simulink model "Test_Display"  (Simulink 8.1)
settings: Solver=ode45  SolverMode=SingleTasking  StartTime=0.0  StopTime=10.0  RelTol=1e-3
undefined symbols (not defined in the file): get, hot
libraries: dspsnks4 x1
(part 2 of 3)

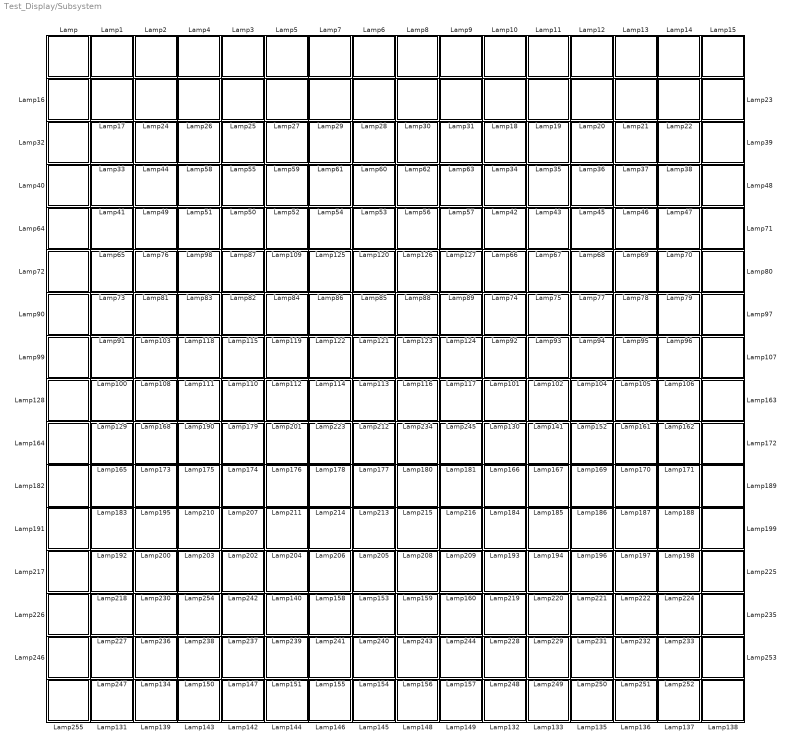
== system Test_Display/Subsystem ==
  Lamp : Subsystem  DialogController=hmiCreateDDGDialog  mask(MWDashboardBlock){webBlockId=edf84850-d0fe-4c8a-86f7-eea0c37b674f, webBlockType=lamp, ShowInLibBrowser=on, ShowInitialText=on, HMISrcModelName=[]}
      mask prompts: webBlockType "WebBlock Type"; HMISrcModelName "Source Model"
      mask Help: helpview([docroot '/mapfiles/simulink.map'], 'hmi_lamp')
      mask Display:
      | if strcmp(get_param(bdroot(gcb),'BlockDiagramType'), 'library')
      |     image([(matlabroot) '/toolbox/simulink/hmi/icons/Lamp.png']);
      | end
  Lamp1 : Subsystem  DialogController=hmiCreateDDGDialog  mask(MWDashboardBlock){webBlockId=fd4cb8b6-599e-465c-bf44-31615dcb3fd4, webBlockType=lamp, ShowInLibBrowser=on, ShowInitialText=on, HMISrcModelName=[]}
      mask prompts: webBlockType "WebBlock Type"; HMISrcModelName "Source Model"
      mask Help: helpview([docroot '/mapfiles/simulink.map'], 'hmi_lamp')
      mask Display:
      | if strcmp(get_param(bdroot(gcb),'BlockDiagramType'), 'library')
      |     image([(matlabroot) '/toolbox/simulink/hmi/icons/Lamp.png']);
      | end
  Lamp10 : Subsystem  DialogController=hmiCreateDDGDialog  mask(MWDashboardBlock){webBlockId=69970134-2694-491f-b422-9ae462ee0038, webBlockType=lamp, ShowInLibBrowser=on, ShowInitialText=on, HMISrcModelName=[]}
      mask prompts: webBlockType "WebBlock Type"; HMISrcModelName "Source Model"
      mask Help: helpview([docroot '/mapfiles/simulink.map'], 'hmi_lamp')
      mask Display:
      | if strcmp(get_param(bdroot(gcb),'BlockDiagramType'), 'library')
      |     image([(matlabroot) '/toolbox/simulink/hmi/icons/Lamp.png']);
      | end
  Lamp100 : Subsystem  DialogController=hmiCreateDDGDialog  mask(MWDashboardBlock){webBlockId=49397023-e76e-4e1f-be5b-ec227a720212, webBlockType=lamp, ShowInLibBrowser=on, ShowInitialText=on, HMISrcModelName=[]}
      mask prompts: webBlockType "WebBlock Type"; HMISrcModelName "Source Model"
      mask Help: helpview([docroot '/mapfiles/simulink.map'], 'hmi_lamp')
      mask Display:
      | if strcmp(get_param(bdroot(gcb),'BlockDiagramType'), 'library')
      |     image([(matlabroot) '/toolbox/simulink/hmi/icons/Lamp.png']);
      | end
  Lamp101 : Subsystem  DialogController=hmiCreateDDGDialog  mask(MWDashboardBlock){webBlockId=21b2a518-b5e8-4574-abab-928d7426710c, webBlockType=lamp, ShowInLibBrowser=on, ShowInitialText=on, HMISrcModelName=[]}
      mask prompts: webBlockType "WebBlock Type"; HMISrcModelName "Source Model"
      mask Help: helpview([docroot '/mapfiles/simulink.map'], 'hmi_lamp')
      mask Display:
      | if strcmp(get_param(bdroot(gcb),'BlockDiagramType'), 'library')
      |     image([(matlabroot) '/toolbox/simulink/hmi/icons/Lamp.png']);
      | end
  Lamp102 : Subsystem  DialogController=hmiCreateDDGDialog  mask(MWDashboardBlock){webBlockId=9ad93c2d-efff-4ac7-a816-7961f3646538, webBlockType=lamp, ShowInLibBrowser=on, ShowInitialText=on, HMISrcModelName=[]}
      mask prompts: webBlockType "WebBlock Type"; HMISrcModelName "Source Model"
      mask Help: helpview([docroot '/mapfiles/simulink.map'], 'hmi_lamp')
      mask Display:
      | if strcmp(get_param(bdroot(gcb),'BlockDiagramType'), 'library')
      |     image([(matlabroot) '/toolbox/simulink/hmi/icons/Lamp.png']);
      | end
  Lamp103 : Subsystem  DialogController=hmiCreateDDGDialog  mask(MWDashboardBlock){webBlockId=b3c12dab-38df-4fcb-add2-5a3df45dc055, webBlockType=lamp, ShowInLibBrowser=on, ShowInitialText=on, HMISrcModelName=[]}
      mask prompts: webBlockType "WebBlock Type"; HMISrcModelName "Source Model"
      mask Help: helpview([docroot '/mapfiles/simulink.map'], 'hmi_lamp')
      mask Display:
      | if strcmp(get_param(bdroot(gcb),'BlockDiagramType'), 'library')
      |     image([(matlabroot) '/toolbox/simulink/hmi/icons/Lamp.png']);
      | end
  Lamp104 : Subsystem  DialogController=hmiCreateDDGDialog  mask(MWDashboardBlock){webBlockId=22654bdc-6924-4c41-873f-0dac80d459c9, webBlockType=lamp, ShowInLibBrowser=on, ShowInitialText=on, HMISrcModelName=[]}
      mask prompts: webBlockType "WebBlock Type"; HMISrcModelName "Source Model"
      mask Help: helpview([docroot '/mapfiles/simulink.map'], 'hmi_lamp')
      mask Display:
      | if strcmp(get_param(bdroot(gcb),'BlockDiagramType'), 'library')
      |     image([(matlabroot) '/toolbox/simulink/hmi/icons/Lamp.png']);
      | end
  Lamp105 : Subsystem  DialogController=hmiCreateDDGDialog  mask(MWDashboardBlock){webBlockId=5a7a78fc-d4e3-496d-b8a8-b493089be8de, webBlockType=lamp, ShowInLibBrowser=on, ShowInitialText=on, HMISrcModelName=[]}
      mask prompts: webBlockType "WebBlock Type"; HMISrcModelName "Source Model"
      mask Help: helpview([docroot '/mapfiles/simulink.map'], 'hmi_lamp')
      mask Display:
      | if strcmp(get_param(bdroot(gcb),'BlockDiagramType'), 'library')
      |     image([(matlabroot) '/toolbox/simulink/hmi/icons/Lamp.png']);
      | end
  Lamp106 : Subsystem  DialogController=hmiCreateDDGDialog  mask(MWDashboardBlock){webBlockId=3a2bc532-a839-46f6-9bbc-20018f0d8f64, webBlockType=lamp, ShowInLibBrowser=on, ShowInitialText=on, HMISrcModelName=[]}
      mask prompts: webBlockType "WebBlock Type"; HMISrcModelName "Source Model"
      mask Help: helpview([docroot '/mapfiles/simulink.map'], 'hmi_lamp')
      mask Display:
      | if strcmp(get_param(bdroot(gcb),'BlockDiagramType'), 'library')
      |     image([(matlabroot) '/toolbox/simulink/hmi/icons/Lamp.png']);
      | end
  Lamp107 : Subsystem  DialogController=hmiCreateDDGDialog  mask(MWDashboardBlock){webBlockId=dba8c154-a909-43bc-b6e3-c0b3528fa1e0, webBlockType=lamp, ShowInLibBrowser=on, ShowInitialText=on, HMISrcModelName=[]}
      mask prompts: webBlockType "WebBlock Type"; HMISrcModelName "Source Model"
      mask Help: helpview([docroot '/mapfiles/simulink.map'], 'hmi_lamp')
      mask Display:
      | if strcmp(get_param(bdroot(gcb),'BlockDiagramType'), 'library')
      |     image([(matlabroot) '/toolbox/simulink/hmi/icons/Lamp.png']);
      | end
  Lamp108 : Subsystem  DialogController=hmiCreateDDGDialog  mask(MWDashboardBlock){webBlockId=a7c0c051-3ddd-4c85-a3d7-890d827bbacd, webBlockType=lamp, ShowInLibBrowser=on, ShowInitialText=on, HMISrcModelName=[]}
      mask prompts: webBlockType "WebBlock Type"; HMISrcModelName "Source Model"
      mask Help: helpview([docroot '/mapfiles/simulink.map'], 'hmi_lamp')
      mask Display:
      | if strcmp(get_param(bdroot(gcb),'BlockDiagramType'), 'library')
      |     image([(matlabroot) '/toolbox/simulink/hmi/icons/Lamp.png']);
      | end
  Lamp109 : Subsystem  DialogController=hmiCreateDDGDialog  mask(MWDashboardBlock){webBlockId=68039627-b65d-475a-b7d3-5dd921e9c6da, webBlockType=lamp, ShowInLibBrowser=on, ShowInitialText=on, HMISrcModelName=[]}
      mask prompts: webBlockType "WebBlock Type"; HMISrcModelName "Source Model"
      mask Help: helpview([docroot '/mapfiles/simulink.map'], 'hmi_lamp')
      mask Display:
      | if strcmp(get_param(bdroot(gcb),'BlockDiagramType'), 'library')
      |     image([(matlabroot) '/toolbox/simulink/hmi/icons/Lamp.png']);
      | end
  Lamp11 : Subsystem  DialogController=hmiCreateDDGDialog  mask(MWDashboardBlock){webBlockId=17d759d2-7a4a-42db-8b8d-8621e0edc736, webBlockType=lamp, ShowInLibBrowser=on, ShowInitialText=on, HMISrcModelName=[]}
      mask prompts: webBlockType "WebBlock Type"; HMISrcModelName "Source Model"
      mask Help: helpview([docroot '/mapfiles/simulink.map'], 'hmi_lamp')
      mask Display:
      | if strcmp(get_param(bdroot(gcb),'BlockDiagramType'), 'library')
      |     image([(matlabroot) '/toolbox/simulink/hmi/icons/Lamp.png']);
      | end
  Lamp110 : Subsystem  DialogController=hmiCreateDDGDialog  mask(MWDashboardBlock){webBlockId=ad71e308-a508-459b-8e0f-4282464f22fe, webBlockType=lamp, ShowInLibBrowser=on, ShowInitialText=on, HMISrcModelName=[]}
      mask prompts: webBlockType "WebBlock Type"; HMISrcModelName "Source Model"
      mask Help: helpview([docroot '/mapfiles/simulink.map'], 'hmi_lamp')
      mask Display:
      | if strcmp(get_param(bdroot(gcb),'BlockDiagramType'), 'library')
      |     image([(matlabroot) '/toolbox/simulink/hmi/icons/Lamp.png']);
      | end
  Lamp111 : Subsystem  DialogController=hmiCreateDDGDialog  mask(MWDashboardBlock){webBlockId=650bb823-101c-407e-9790-47f3807fb796, webBlockType=lamp, ShowInLibBrowser=on, ShowInitialText=on, HMISrcModelName=[]}
      mask prompts: webBlockType "WebBlock Type"; HMISrcModelName "Source Model"
      mask Help: helpview([docroot '/mapfiles/simulink.map'], 'hmi_lamp')
      mask Display:
      | if strcmp(get_param(bdroot(gcb),'BlockDiagramType'), 'library')
      |     image([(matlabroot) '/toolbox/simulink/hmi/icons/Lamp.png']);
      | end
  Lamp112 : Subsystem  DialogController=hmiCreateDDGDialog  mask(MWDashboardBlock){webBlockId=423ee99d-c28c-43df-a12a-3af234ac6943, webBlockType=lamp, ShowInLibBrowser=on, ShowInitialText=on, HMISrcModelName=[]}
      mask prompts: webBlockType "WebBlock Type"; HMISrcModelName "Source Model"
      mask Help: helpview([docroot '/mapfiles/simulink.map'], 'hmi_lamp')
      mask Display:
      | if strcmp(get_param(bdroot(gcb),'BlockDiagramType'), 'library')
      |     image([(matlabroot) '/toolbox/simulink/hmi/icons/Lamp.png']);
      | end
  Lamp113 : Subsystem  DialogController=hmiCreateDDGDialog  mask(MWDashboardBlock){webBlockId=1a9c237c-8958-40c1-8183-6b5bf75441e2, webBlockType=lamp, ShowInLibBrowser=on, ShowInitialText=on, HMISrcModelName=[]}
      mask prompts: webBlockType "WebBlock Type"; HMISrcModelName "Source Model"
      mask Help: helpview([docroot '/mapfiles/simulink.map'], 'hmi_lamp')
      mask Display:
      | if strcmp(get_param(bdroot(gcb),'BlockDiagramType'), 'library')
      |     image([(matlabroot) '/toolbox/simulink/hmi/icons/Lamp.png']);
      | end
  Lamp114 : Subsystem  DialogController=hmiCreateDDGDialog  mask(MWDashboardBlock){webBlockId=59713dff-163f-48a3-89de-46bb5d4dd39c, webBlockType=lamp, ShowInLibBrowser=on, ShowInitialText=on, HMISrcModelName=[]}
      mask prompts: webBlockType "WebBlock Type"; HMISrcModelName "Source Model"
      mask Help: helpview([docroot '/mapfiles/simulink.map'], 'hmi_lamp')
      mask Display:
      | if strcmp(get_param(bdroot(gcb),'BlockDiagramType'), 'library')
      |     image([(matlabroot) '/toolbox/simulink/hmi/icons/Lamp.png']);
      | end
  Lamp115 : Subsystem  DialogController=hmiCreateDDGDialog  mask(MWDashboardBlock){webBlockId=ca91e4aa-4a84-4aef-8eff-59d3ab8b4ed0, webBlockType=lamp, ShowInLibBrowser=on, ShowInitialText=on, HMISrcModelName=[]}
      mask prompts: webBlockType "WebBlock Type"; HMISrcModelName "Source Model"
      mask Help: helpview([docroot '/mapfiles/simulink.map'], 'hmi_lamp')
      mask Display:
      | if strcmp(get_param(bdroot(gcb),'BlockDiagramType'), 'library')
      |     image([(matlabroot) '/toolbox/simulink/hmi/icons/Lamp.png']);
      | end
  Lamp116 : Subsystem  DialogController=hmiCreateDDGDialog  mask(MWDashboardBlock){webBlockId=ea0446a5-980a-44d1-baf7-efdbd4c4c0cf, webBlockType=lamp, ShowInLibBrowser=on, ShowInitialText=on, HMISrcModelName=[]}
      mask prompts: webBlockType "WebBlock Type"; HMISrcModelName "Source Model"
      mask Help: helpview([docroot '/mapfiles/simulink.map'], 'hmi_lamp')
      mask Display:
      | if strcmp(get_param(bdroot(gcb),'BlockDiagramType'), 'library')
      |     image([(matlabroot) '/toolbox/simulink/hmi/icons/Lamp.png']);
      | end
  Lamp117 : Subsystem  DialogController=hmiCreateDDGDialog  mask(MWDashboardBlock){webBlockId=6f6da4d9-b8fd-41db-ad2e-5eafed5489c3, webBlockType=lamp, ShowInLibBrowser=on, ShowInitialText=on, HMISrcModelName=[]}
      mask prompts: webBlockType "WebBlock Type"; HMISrcModelName "Source Model"
      mask Help: helpview([docroot '/mapfiles/simulink.map'], 'hmi_lamp')
      mask Display:
      | if strcmp(get_param(bdroot(gcb),'BlockDiagramType'), 'library')
      |     image([(matlabroot) '/toolbox/simulink/hmi/icons/Lamp.png']);
      | end
  Lamp118 : Subsystem  DialogController=hmiCreateDDGDialog  mask(MWDashboardBlock){webBlockId=a4cd4763-fce0-4138-a61c-a9eaa5240dcf, webBlockType=lamp, ShowInLibBrowser=on, ShowInitialText=on, HMISrcModelName=[]}
      mask prompts: webBlockType "WebBlock Type"; HMISrcModelName "Source Model"
      mask Help: helpview([docroot '/mapfiles/simulink.map'], 'hmi_lamp')
      mask Display:
      | if strcmp(get_param(bdroot(gcb),'BlockDiagramType'), 'library')
      |     image([(matlabroot) '/toolbox/simulink/hmi/icons/Lamp.png']);
      | end
  Lamp119 : Subsystem  DialogController=hmiCreateDDGDialog  mask(MWDashboardBlock){webBlockId=e5efb401-ac08-44a6-bfd0-4540585fee9a, webBlockType=lamp, ShowInLibBrowser=on, ShowInitialText=on, HMISrcModelName=[]}
      mask prompts: webBlockType "WebBlock Type"; HMISrcModelName "Source Model"
      mask Help: helpview([docroot '/mapfiles/simulink.map'], 'hmi_lamp')
      mask Display:
      | if strcmp(get_param(bdroot(gcb),'BlockDiagramType'), 'library')
      |     image([(matlabroot) '/toolbox/simulink/hmi/icons/Lamp.png']);
      | end
  Lamp12 : Subsystem  DialogController=hmiCreateDDGDialog  mask(MWDashboardBlock){webBlockId=2739aeb3-55c9-4fba-ad1b-ffe4ed783479, webBlockType=lamp, ShowInLibBrowser=on, ShowInitialText=on, HMISrcModelName=[]}
      mask prompts: webBlockType "WebBlock Type"; HMISrcModelName "Source Model"
      mask Help: helpview([docroot '/mapfiles/simulink.map'], 'hmi_lamp')
      mask Display:
      | if strcmp(get_param(bdroot(gcb),'BlockDiagramType'), 'library')
      |     image([(matlabroot) '/toolbox/simulink/hmi/icons/Lamp.png']);
      | end
  Lamp120 : Subsystem  DialogController=hmiCreateDDGDialog  mask(MWDashboardBlock){webBlockId=4de6be70-ca78-43c6-a822-f9fd70f81b9a, webBlockType=lamp, ShowInLibBrowser=on, ShowInitialText=on, HMISrcModelName=[]}
      mask prompts: webBlockType "WebBlock Type"; HMISrcModelName "Source Model"
      mask Help: helpview([docroot '/mapfiles/simulink.map'], 'hmi_lamp')
      mask Display:
      | if strcmp(get_param(bdroot(gcb),'BlockDiagramType'), 'library')
      |     image([(matlabroot) '/toolbox/simulink/hmi/icons/Lamp.png']);
      | end
  Lamp121 : Subsystem  DialogController=hmiCreateDDGDialog  mask(MWDashboardBlock){webBlockId=ec3c07a6-ed4f-446b-a6db-729d5e1aac5e, webBlockType=lamp, ShowInLibBrowser=on, ShowInitialText=on, HMISrcModelName=[]}
      mask prompts: webBlockType "WebBlock Type"; HMISrcModelName "Source Model"
      mask Help: helpview([docroot '/mapfiles/simulink.map'], 'hmi_lamp')
      mask Display:
      | if strcmp(get_param(bdroot(gcb),'BlockDiagramType'), 'library')
      |     image([(matlabroot) '/toolbox/simulink/hmi/icons/Lamp.png']);
      | end
  Lamp122 : Subsystem  DialogController=hmiCreateDDGDialog  mask(MWDashboardBlock){webBlockId=6e468738-635a-42dc-b04e-3cbfa3067652, webBlockType=lamp, ShowInLibBrowser=on, ShowInitialText=on, HMISrcModelName=[]}
      mask prompts: webBlockType "WebBlock Type"; HMISrcModelName "Source Model"
      mask Help: helpview([docroot '/mapfiles/simulink.map'], 'hmi_lamp')
      mask Display:
      | if strcmp(get_param(bdroot(gcb),'BlockDiagramType'), 'library')
      |     image([(matlabroot) '/toolbox/simulink/hmi/icons/Lamp.png']);
      | end
  Lamp123 : Subsystem  DialogController=hmiCreateDDGDialog  mask(MWDashboardBlock){webBlockId=fb95ced1-5fd5-4dd6-99a4-486117cc7b04, webBlockType=lamp, ShowInLibBrowser=on, ShowInitialText=on, HMISrcModelName=[]}
      mask prompts: webBlockType "WebBlock Type"; HMISrcModelName "Source Model"
      mask Help: helpview([docroot '/mapfiles/simulink.map'], 'hmi_lamp')
      mask Display:
      | if strcmp(get_param(bdroot(gcb),'BlockDiagramType'), 'library')
      |     image([(matlabroot) '/toolbox/simulink/hmi/icons/Lamp.png']);
      | end
  Lamp124 : Subsystem  DialogController=hmiCreateDDGDialog  mask(MWDashboardBlock){webBlockId=8cc34a89-169c-45fb-add0-c245fffb35f4, webBlockType=lamp, ShowInLibBrowser=on, ShowInitialText=on, HMISrcModelName=[]}
      mask prompts: webBlockType "WebBlock Type"; HMISrcModelName "Source Model"
      mask Help: helpview([docroot '/mapfiles/simulink.map'], 'hmi_lamp')
      mask Display:
      | if strcmp(get_param(bdroot(gcb),'BlockDiagramType'), 'library')
      |     image([(matlabroot) '/toolbox/simulink/hmi/icons/Lamp.png']);
      | end
  Lamp125 : Subsystem  DialogController=hmiCreateDDGDialog  mask(MWDashboardBlock){webBlockId=5e75099f-bab6-47c8-9d5a-45cdd18ada81, webBlockType=lamp, ShowInLibBrowser=on, ShowInitialText=on, HMISrcModelName=[]}
      mask prompts: webBlockType "WebBlock Type"; HMISrcModelName "Source Model"
      mask Help: helpview([docroot '/mapfiles/simulink.map'], 'hmi_lamp')
      mask Display:
      | if strcmp(get_param(bdroot(gcb),'BlockDiagramType'), 'library')
      |     image([(matlabroot) '/toolbox/simulink/hmi/icons/Lamp.png']);
      | end
  Lamp126 : Subsystem  DialogController=hmiCreateDDGDialog  mask(MWDashboardBlock){webBlockId=b24af4a7-3b56-44e6-9307-9233d0605101, webBlockType=lamp, ShowInLibBrowser=on, ShowInitialText=on, HMISrcModelName=[]}
      mask prompts: webBlockType "WebBlock Type"; HMISrcModelName "Source Model"
      mask Help: helpview([docroot '/mapfiles/simulink.map'], 'hmi_lamp')
      mask Display:
      | if strcmp(get_param(bdroot(gcb),'BlockDiagramType'), 'library')
      |     image([(matlabroot) '/toolbox/simulink/hmi/icons/Lamp.png']);
      | end
  Lamp127 : Subsystem  DialogController=hmiCreateDDGDialog  mask(MWDashboardBlock){webBlockId=f9e12296-8670-4a96-b8dc-f227c20c59c8, webBlockType=lamp, ShowInLibBrowser=on, ShowInitialText=on, HMISrcModelName=[]}
      mask prompts: webBlockType "WebBlock Type"; HMISrcModelName "Source Model"
      mask Help: helpview([docroot '/mapfiles/simulink.map'], 'hmi_lamp')
      mask Display:
      | if strcmp(get_param(bdroot(gcb),'BlockDiagramType'), 'library')
      |     image([(matlabroot) '/toolbox/simulink/hmi/icons/Lamp.png']);
      | end
  Lamp128 : Subsystem  DialogController=hmiCreateDDGDialog  mask(MWDashboardBlock){webBlockId=639b4a5e-2d2b-4481-a81d-53f4802d670a, webBlockType=lamp, ShowInLibBrowser=on, ShowInitialText=on, HMISrcModelName=[]}
      mask prompts: webBlockType "WebBlock Type"; HMISrcModelName "Source Model"
      mask Help: helpview([docroot '/mapfiles/simulink.map'], 'hmi_lamp')
      mask Display:
      | if strcmp(get_param(bdroot(gcb),'BlockDiagramType'), 'library')
      |     image([(matlabroot) '/toolbox/simulink/hmi/icons/Lamp.png']);
      | end
  Lamp129 : Subsystem  DialogController=hmiCreateDDGDialog  mask(MWDashboardBlock){webBlockId=2bbac042-df92-44e2-886a-26cf5aa8e5a7, webBlockType=lamp, ShowInLibBrowser=on, ShowInitialText=on, HMISrcModelName=[]}
      mask prompts: webBlockType "WebBlock Type"; HMISrcModelName "Source Model"
      mask Help: helpview([docroot '/mapfiles/simulink.map'], 'hmi_lamp')
      mask Display:
      | if strcmp(get_param(bdroot(gcb),'BlockDiagramType'), 'library')
      |     image([(matlabroot) '/toolbox/simulink/hmi/icons/Lamp.png']);
      | end
  Lamp13 : Subsystem  DialogController=hmiCreateDDGDialog  mask(MWDashboardBlock){webBlockId=10de76a9-a845-4e5b-a06c-3d4b0e136d3c, webBlockType=lamp, ShowInLibBrowser=on, ShowInitialText=on, HMISrcModelName=[]}
      mask prompts: webBlockType "WebBlock Type"; HMISrcModelName "Source Model"
      mask Help: helpview([docroot '/mapfiles/simulink.map'], 'hmi_lamp')
      mask Display:
      | if strcmp(get_param(bdroot(gcb),'BlockDiagramType'), 'library')
      |     image([(matlabroot) '/toolbox/simulink/hmi/icons/Lamp.png']);
      | end
  Lamp130 : Subsystem  DialogController=hmiCreateDDGDialog  mask(MWDashboardBlock){webBlockId=03246cb9-1490-4c04-bce7-8577a1ad03d9, webBlockType=lamp, ShowInLibBrowser=on, ShowInitialText=on, HMISrcModelName=[]}
      mask prompts: webBlockType "WebBlock Type"; HMISrcModelName "Source Model"
      mask Help: helpview([docroot '/mapfiles/simulink.map'], 'hmi_lamp')
      mask Display:
      | if strcmp(get_param(bdroot(gcb),'BlockDiagramType'), 'library')
      |     image([(matlabroot) '/toolbox/simulink/hmi/icons/Lamp.png']);
      | end
  Lamp131 : Subsystem  DialogController=hmiCreateDDGDialog  mask(MWDashboardBlock){webBlockId=bc19434d-be49-4c90-9f4f-d30ae243e62e, webBlockType=lamp, ShowInLibBrowser=on, ShowInitialText=on, HMISrcModelName=[]}
      mask prompts: webBlockType "WebBlock Type"; HMISrcModelName "Source Model"
      mask Help: helpview([docroot '/mapfiles/simulink.map'], 'hmi_lamp')
      mask Display:
      | if strcmp(get_param(bdroot(gcb),'BlockDiagramType'), 'library')
      |     image([(matlabroot) '/toolbox/simulink/hmi/icons/Lamp.png']);
      | end
  Lamp132 : Subsystem  DialogController=hmiCreateDDGDialog  mask(MWDashboardBlock){webBlockId=69249e84-f16d-4676-be2b-d7059b0a9994, webBlockType=lamp, ShowInLibBrowser=on, ShowInitialText=on, HMISrcModelName=[]}
      mask prompts: webBlockType "WebBlock Type"; HMISrcModelName "Source Model"
      mask Help: helpview([docroot '/mapfiles/simulink.map'], 'hmi_lamp')
      mask Display:
      | if strcmp(get_param(bdroot(gcb),'BlockDiagramType'), 'library')
      |     image([(matlabroot) '/toolbox/simulink/hmi/icons/Lamp.png']);
      | end
  Lamp133 : Subsystem  DialogController=hmiCreateDDGDialog  mask(MWDashboardBlock){webBlockId=a551e0c3-b966-4766-ba83-f6a20ae4271b, webBlockType=lamp, ShowInLibBrowser=on, ShowInitialText=on, HMISrcModelName=[]}
      mask prompts: webBlockType "WebBlock Type"; HMISrcModelName "Source Model"
      mask Help: helpview([docroot '/mapfiles/simulink.map'], 'hmi_lamp')
      mask Display:
      | if strcmp(get_param(bdroot(gcb),'BlockDiagramType'), 'library')
      |     image([(matlabroot) '/toolbox/simulink/hmi/icons/Lamp.png']);
      | end
  Lamp134 : Subsystem  DialogController=hmiCreateDDGDialog  mask(MWDashboardBlock){webBlockId=9226dd28-2f61-4cbc-916d-2f003ff13875, webBlockType=lamp, ShowInLibBrowser=on, ShowInitialText=on, HMISrcModelName=[]}
      mask prompts: webBlockType "WebBlock Type"; HMISrcModelName "Source Model"
      mask Help: helpview([docroot '/mapfiles/simulink.map'], 'hmi_lamp')
      mask Display:
      | if strcmp(get_param(bdroot(gcb),'BlockDiagramType'), 'library')
      |     image([(matlabroot) '/toolbox/simulink/hmi/icons/Lamp.png']);
      | end
  Lamp135 : Subsystem  DialogController=hmiCreateDDGDialog  mask(MWDashboardBlock){webBlockId=30756550-dc76-4560-be15-4ef60ec92a06, webBlockType=lamp, ShowInLibBrowser=on, ShowInitialText=on, HMISrcModelName=[]}
      mask prompts: webBlockType "WebBlock Type"; HMISrcModelName "Source Model"
      mask Help: helpview([docroot '/mapfiles/simulink.map'], 'hmi_lamp')
      mask Display:
      | if strcmp(get_param(bdroot(gcb),'BlockDiagramType'), 'library')
      |     image([(matlabroot) '/toolbox/simulink/hmi/icons/Lamp.png']);
      | end
  Lamp136 : Subsystem  DialogController=hmiCreateDDGDialog  mask(MWDashboardBlock){webBlockId=03fb90b9-30b9-4fc6-9e3f-ec2903734866, webBlockType=lamp, ShowInLibBrowser=on, ShowInitialText=on, HMISrcModelName=[]}
      mask prompts: webBlockType "WebBlock Type"; HMISrcModelName "Source Model"
      mask Help: helpview([docroot '/mapfiles/simulink.map'], 'hmi_lamp')
      mask Display:
      | if strcmp(get_param(bdroot(gcb),'BlockDiagramType'), 'library')
      |     image([(matlabroot) '/toolbox/simulink/hmi/icons/Lamp.png']);
      | end
  Lamp137 : Subsystem  DialogController=hmiCreateDDGDialog  mask(MWDashboardBlock){webBlockId=feb07395-20a8-4e13-b12c-940a4c08d7e3, webBlockType=lamp, ShowInLibBrowser=on, ShowInitialText=on, HMISrcModelName=[]}
      mask prompts: webBlockType "WebBlock Type"; HMISrcModelName "Source Model"
      mask Help: helpview([docroot '/mapfiles/simulink.map'], 'hmi_lamp')
      mask Display:
      | if strcmp(get_param(bdroot(gcb),'BlockDiagramType'), 'library')
      |     image([(matlabroot) '/toolbox/simulink/hmi/icons/Lamp.png']);
      | end
  Lamp138 : Subsystem  DialogController=hmiCreateDDGDialog  mask(MWDashboardBlock){webBlockId=e67aa3ec-cb25-4e0a-b9fe-ecabe559c076, webBlockType=lamp, ShowInLibBrowser=on, ShowInitialText=on, HMISrcModelName=[]}
      mask prompts: webBlockType "WebBlock Type"; HMISrcModelName "Source Model"
      mask Help: helpview([docroot '/mapfiles/simulink.map'], 'hmi_lamp')
      mask Display:
      | if strcmp(get_param(bdroot(gcb),'BlockDiagramType'), 'library')
      |     image([(matlabroot) '/toolbox/simulink/hmi/icons/Lamp.png']);
      | end
  Lamp139 : Subsystem  DialogController=hmiCreateDDGDialog  mask(MWDashboardBlock){webBlockId=5702d281-6869-40e3-983b-7b49f3856835, webBlockType=lamp, ShowInLibBrowser=on, ShowInitialText=on, HMISrcModelName=[]}
      mask prompts: webBlockType "WebBlock Type"; HMISrcModelName "Source Model"
      mask Help: helpview([docroot '/mapfiles/simulink.map'], 'hmi_lamp')
      mask Display:
      | if strcmp(get_param(bdroot(gcb),'BlockDiagramType'), 'library')
      |     image([(matlabroot) '/toolbox/simulink/hmi/icons/Lamp.png']);
      | end
  Lamp14 : Subsystem  DialogController=hmiCreateDDGDialog  mask(MWDashboardBlock){webBlockId=52bcf478-ee21-4e59-a68c-c7f4a2aa98d0, webBlockType=lamp, ShowInLibBrowser=on, ShowInitialText=on, HMISrcModelName=[]}
      mask prompts: webBlockType "WebBlock Type"; HMISrcModelName "Source Model"
      mask Help: helpview([docroot '/mapfiles/simulink.map'], 'hmi_lamp')
      mask Display:
      | if strcmp(get_param(bdroot(gcb),'BlockDiagramType'), 'library')
      |     image([(matlabroot) '/toolbox/simulink/hmi/icons/Lamp.png']);
      | end
  Lamp140 : Subsystem  DialogController=hmiCreateDDGDialog  mask(MWDashboardBlock){webBlockId=c8ddbf31-eec6-4f92-8498-7ef8840ee0c5, webBlockType=lamp, ShowInLibBrowser=on, ShowInitialText=on, HMISrcModelName=[]}
      mask prompts: webBlockType "WebBlock Type"; HMISrcModelName "Source Model"
      mask Help: helpview([docroot '/mapfiles/simulink.map'], 'hmi_lamp')
      mask Display:
      | if strcmp(get_param(bdroot(gcb),'BlockDiagramType'), 'library')
      |     image([(matlabroot) '/toolbox/simulink/hmi/icons/Lamp.png']);
      | end
  Lamp141 : Subsystem  DialogController=hmiCreateDDGDialog  mask(MWDashboardBlock){webBlockId=41c5764a-9e06-4781-a764-558b60c73110, webBlockType=lamp, ShowInLibBrowser=on, ShowInitialText=on, HMISrcModelName=[]}
      mask prompts: webBlockType "WebBlock Type"; HMISrcModelName "Source Model"
      mask Help: helpview([docroot '/mapfiles/simulink.map'], 'hmi_lamp')
      mask Display:
      | if strcmp(get_param(bdroot(gcb),'BlockDiagramType'), 'library')
      |     image([(matlabroot) '/toolbox/simulink/hmi/icons/Lamp.png']);
      | end
  Lamp142 : Subsystem  DialogController=hmiCreateDDGDialog  mask(MWDashboardBlock){webBlockId=7e472b11-54a6-4a14-92de-30822cdd07d8, webBlockType=lamp, ShowInLibBrowser=on, ShowInitialText=on, HMISrcModelName=[]}
      mask prompts: webBlockType "WebBlock Type"; HMISrcModelName "Source Model"
      mask Help: helpview([docroot '/mapfiles/simulink.map'], 'hmi_lamp')
      mask Display:
      | if strcmp(get_param(bdroot(gcb),'BlockDiagramType'), 'library')
      |     image([(matlabroot) '/toolbox/simulink/hmi/icons/Lamp.png']);
      | end
  Lamp143 : Subsystem  DialogController=hmiCreateDDGDialog  mask(MWDashboardBlock){webBlockId=bcc07bfa-ec91-4a12-bfd0-1db324e1536c, webBlockType=lamp, ShowInLibBrowser=on, ShowInitialText=on, HMISrcModelName=[]}
      mask prompts: webBlockType "WebBlock Type"; HMISrcModelName "Source Model"
      mask Help: helpview([docroot '/mapfiles/simulink.map'], 'hmi_lamp')
      mask Display:
      | if strcmp(get_param(bdroot(gcb),'BlockDiagramType'), 'library')
      |     image([(matlabroot) '/toolbox/simulink/hmi/icons/Lamp.png']);
      | end
  Lamp144 : Subsystem  DialogController=hmiCreateDDGDialog  mask(MWDashboardBlock){webBlockId=27548a7b-adaa-421d-8d7b-188519919b59, webBlockType=lamp, ShowInLibBrowser=on, ShowInitialText=on, HMISrcModelName=[]}
      mask prompts: webBlockType "WebBlock Type"; HMISrcModelName "Source Model"
      mask Help: helpview([docroot '/mapfiles/simulink.map'], 'hmi_lamp')
      mask Display:
      | if strcmp(get_param(bdroot(gcb),'BlockDiagramType'), 'library')
      |     image([(matlabroot) '/toolbox/simulink/hmi/icons/Lamp.png']);
      | end
  Lamp145 : Subsystem  DialogController=hmiCreateDDGDialog  mask(MWDashboardBlock){webBlockId=71c8b46b-6630-4274-8b1f-017c479c4682, webBlockType=lamp, ShowInLibBrowser=on, ShowInitialText=on, HMISrcModelName=[]}
      mask prompts: webBlockType "WebBlock Type"; HMISrcModelName "Source Model"
      mask Help: helpview([docroot '/mapfiles/simulink.map'], 'hmi_lamp')
      mask Display:
      | if strcmp(get_param(bdroot(gcb),'BlockDiagramType'), 'library')
      |     image([(matlabroot) '/toolbox/simulink/hmi/icons/Lamp.png']);
      | end
  Lamp146 : Subsystem  DialogController=hmiCreateDDGDialog  mask(MWDashboardBlock){webBlockId=926c75ad-6279-403e-b3a2-13e7804491cf, webBlockType=lamp, ShowInLibBrowser=on, ShowInitialText=on, HMISrcModelName=[]}
      mask prompts: webBlockType "WebBlock Type"; HMISrcModelName "Source Model"
      mask Help: helpview([docroot '/mapfiles/simulink.map'], 'hmi_lamp')
      mask Display:
      | if strcmp(get_param(bdroot(gcb),'BlockDiagramType'), 'library')
      |     image([(matlabroot) '/toolbox/simulink/hmi/icons/Lamp.png']);
      | end
  Lamp147 : Subsystem  DialogController=hmiCreateDDGDialog  mask(MWDashboardBlock){webBlockId=16891fd5-6060-41ae-ace8-865b03101884, webBlockType=lamp, ShowInLibBrowser=on, ShowInitialText=on, HMISrcModelName=[]}
      mask prompts: webBlockType "WebBlock Type"; HMISrcModelName "Source Model"
      mask Help: helpview([docroot '/mapfiles/simulink.map'], 'hmi_lamp')
      mask Display:
      | if strcmp(get_param(bdroot(gcb),'BlockDiagramType'), 'library')
      |     image([(matlabroot) '/toolbox/simulink/hmi/icons/Lamp.png']);
      | end
  Lamp148 : Subsystem  DialogController=hmiCreateDDGDialog  mask(MWDashboardBlock){webBlockId=50d56bf2-3d5a-464c-af77-29868d3b584b, webBlockType=lamp, ShowInLibBrowser=on, ShowInitialText=on, HMISrcModelName=[]}
      mask prompts: webBlockType "WebBlock Type"; HMISrcModelName "Source Model"
      mask Help: helpview([docroot '/mapfiles/simulink.map'], 'hmi_lamp')
      mask Display:
      | if strcmp(get_param(bdroot(gcb),'BlockDiagramType'), 'library')
      |     image([(matlabroot) '/toolbox/simulink/hmi/icons/Lamp.png']);
      | end
  Lamp149 : Subsystem  DialogController=hmiCreateDDGDialog  mask(MWDashboardBlock){webBlockId=5c5095b5-6cb5-4f34-ab57-964487ff9750, webBlockType=lamp, ShowInLibBrowser=on, ShowInitialText=on, HMISrcModelName=[]}
      mask prompts: webBlockType "WebBlock Type"; HMISrcModelName "Source Model"
      mask Help: helpview([docroot '/mapfiles/simulink.map'], 'hmi_lamp')
      mask Display:
      | if strcmp(get_param(bdroot(gcb),'BlockDiagramType'), 'library')
      |     image([(matlabroot) '/toolbox/simulink/hmi/icons/Lamp.png']);
      | end
  Lamp15 : Subsystem  DialogController=hmiCreateDDGDialog  mask(MWDashboardBlock){webBlockId=fd6a1799-aaa5-4209-887b-91af1873a865, webBlockType=lamp, ShowInLibBrowser=on, ShowInitialText=on, HMISrcModelName=[]}
      mask prompts: webBlockType "WebBlock Type"; HMISrcModelName "Source Model"
      mask Help: helpview([docroot '/mapfiles/simulink.map'], 'hmi_lamp')
      mask Display:
      | if strcmp(get_param(bdroot(gcb),'BlockDiagramType'), 'library')
      |     image([(matlabroot) '/toolbox/simulink/hmi/icons/Lamp.png']);
      | end
  Lamp150 : Subsystem  DialogController=hmiCreateDDGDialog  mask(MWDashboardBlock){webBlockId=2da9fa6b-7baf-4c14-adac-213ddce0fd6b, webBlockType=lamp, ShowInLibBrowser=on, ShowInitialText=on, HMISrcModelName=[]}
      mask prompts: webBlockType "WebBlock Type"; HMISrcModelName "Source Model"
      mask Help: helpview([docroot '/mapfiles/simulink.map'], 'hmi_lamp')
      mask Display:
      | if strcmp(get_param(bdroot(gcb),'BlockDiagramType'), 'library')
      |     image([(matlabroot) '/toolbox/simulink/hmi/icons/Lamp.png']);
      | end
  Lamp151 : Subsystem  DialogController=hmiCreateDDGDialog  mask(MWDashboardBlock){webBlockId=6527e29f-eb80-49b7-a10c-da95c934fad0, webBlockType=lamp, ShowInLibBrowser=on, ShowInitialText=on, HMISrcModelName=[]}
      mask prompts: webBlockType "WebBlock Type"; HMISrcModelName "Source Model"
      mask Help: helpview([docroot '/mapfiles/simulink.map'], 'hmi_lamp')
      mask Display:
      | if strcmp(get_param(bdroot(gcb),'BlockDiagramType'), 'library')
      |     image([(matlabroot) '/toolbox/simulink/hmi/icons/Lamp.png']);
      | end
  Lamp152 : Subsystem  DialogController=hmiCreateDDGDialog  mask(MWDashboardBlock){webBlockId=650a1d02-f55d-49cc-bfe7-5dfa2b4072b8, webBlockType=lamp, ShowInLibBrowser=on, ShowInitialText=on, HMISrcModelName=[]}
      mask prompts: webBlockType "WebBlock Type"; HMISrcModelName "Source Model"
      mask Help: helpview([docroot '/mapfiles/simulink.map'], 'hmi_lamp')
      mask Display:
      | if strcmp(get_param(bdroot(gcb),'BlockDiagramType'), 'library')
      |     image([(matlabroot) '/toolbox/simulink/hmi/icons/Lamp.png']);
      | end
  Lamp153 : Subsystem  DialogController=hmiCreateDDGDialog  mask(MWDashboardBlock){webBlockId=3b0d2e77-26d1-46f4-a649-06b67f0886c4, webBlockType=lamp, ShowInLibBrowser=on, ShowInitialText=on, HMISrcModelName=[]}
      mask prompts: webBlockType "WebBlock Type"; HMISrcModelName "Source Model"
      mask Help: helpview([docroot '/mapfiles/simulink.map'], 'hmi_lamp')
      mask Display:
      | if strcmp(get_param(bdroot(gcb),'BlockDiagramType'), 'library')
      |     image([(matlabroot) '/toolbox/simulink/hmi/icons/Lamp.png']);
      | end
  Lamp154 : Subsystem  DialogController=hmiCreateDDGDialog  mask(MWDashboardBlock){webBlockId=dbd06766-f249-48d3-aa3b-08955420d0c9, webBlockType=lamp, ShowInLibBrowser=on, ShowInitialText=on, HMISrcModelName=[]}
      mask prompts: webBlockType "WebBlock Type"; HMISrcModelName "Source Model"
      mask Help: helpview([docroot '/mapfiles/simulink.map'], 'hmi_lamp')
      mask Display:
      | if strcmp(get_param(bdroot(gcb),'BlockDiagramType'), 'library')
      |     image([(matlabroot) '/toolbox/simulink/hmi/icons/Lamp.png']);
      | end
  Lamp155 : Subsystem  DialogController=hmiCreateDDGDialog  mask(MWDashboardBlock){webBlockId=ee62f822-f81e-4fe7-9b67-548d6e40486a, webBlockType=lamp, ShowInLibBrowser=on, ShowInitialText=on, HMISrcModelName=[]}
      mask prompts: webBlockType "WebBlock Type"; HMISrcModelName "Source Model"
      mask Help: helpview([docroot '/mapfiles/simulink.map'], 'hmi_lamp')
      mask Display:
      | if strcmp(get_param(bdroot(gcb),'BlockDiagramType'), 'library')
      |     image([(matlabroot) '/toolbox/simulink/hmi/icons/Lamp.png']);
      | end
  Lamp156 : Subsystem  DialogController=hmiCreateDDGDialog  mask(MWDashboardBlock){webBlockId=94100789-9974-499d-9b0a-e57dd5135721, webBlockType=lamp, ShowInLibBrowser=on, ShowInitialText=on, HMISrcModelName=[]}
      mask prompts: webBlockType "WebBlock Type"; HMISrcModelName "Source Model"
      mask Help: helpview([docroot '/mapfiles/simulink.map'], 'hmi_lamp')
      mask Display:
      | if strcmp(get_param(bdroot(gcb),'BlockDiagramType'), 'library')
      |     image([(matlabroot) '/toolbox/simulink/hmi/icons/Lamp.png']);
      | end
  Lamp157 : Subsystem  DialogController=hmiCreateDDGDialog  mask(MWDashboardBlock){webBlockId=7781c26c-5d4e-4256-aa4c-991fed1d4af8, webBlockType=lamp, ShowInLibBrowser=on, ShowInitialText=on, HMISrcModelName=[]}
      mask prompts: webBlockType "WebBlock Type"; HMISrcModelName "Source Model"
      mask Help: helpview([docroot '/mapfiles/simulink.map'], 'hmi_lamp')
      mask Display:
      | if strcmp(get_param(bdroot(gcb),'BlockDiagramType'), 'library')
      |     image([(matlabroot) '/toolbox/simulink/hmi/icons/Lamp.png']);
      | end
  Lamp158 : Subsystem  DialogController=hmiCreateDDGDialog  mask(MWDashboardBlock){webBlockId=30a713e5-f699-42c2-a5fc-3e074a190ced, webBlockType=lamp, ShowInLibBrowser=on, ShowInitialText=on, HMISrcModelName=[]}
      mask prompts: webBlockType "WebBlock Type"; HMISrcModelName "Source Model"
      mask Help: helpview([docroot '/mapfiles/simulink.map'], 'hmi_lamp')
      mask Display:
      | if strcmp(get_param(bdroot(gcb),'BlockDiagramType'), 'library')
      |     image([(matlabroot) '/toolbox/simulink/hmi/icons/Lamp.png']);
      | end
  Lamp159 : Subsystem  DialogController=hmiCreateDDGDialog  mask(MWDashboardBlock){webBlockId=a6c95aee-2192-4b96-b429-370230b93df7, webBlockType=lamp, ShowInLibBrowser=on, ShowInitialText=on, HMISrcModelName=[]}
      mask prompts: webBlockType "WebBlock Type"; HMISrcModelName "Source Model"
      mask Help: helpview([docroot '/mapfiles/simulink.map'], 'hmi_lamp')
      mask Display:
      | if strcmp(get_param(bdroot(gcb),'BlockDiagramType'), 'library')
      |     image([(matlabroot) '/toolbox/simulink/hmi/icons/Lamp.png']);
      | end
  Lamp16 : Subsystem  DialogController=hmiCreateDDGDialog  mask(MWDashboardBlock){webBlockId=540d69e0-b843-4e96-acff-22dc7f87c607, webBlockType=lamp, ShowInLibBrowser=on, ShowInitialText=on, HMISrcModelName=[]}
      mask prompts: webBlockType "WebBlock Type"; HMISrcModelName "Source Model"
      mask Help: helpview([docroot '/mapfiles/simulink.map'], 'hmi_lamp')
      mask Display:
      | if strcmp(get_param(bdroot(gcb),'BlockDiagramType'), 'library')
      |     image([(matlabroot) '/toolbox/simulink/hmi/icons/Lamp.png']);
      | end
  Lamp160 : Subsystem  DialogController=hmiCreateDDGDialog  mask(MWDashboardBlock){webBlockId=0e50a153-1379-4744-be8c-9fe88147fac6, webBlockType=lamp, ShowInLibBrowser=on, ShowInitialText=on, HMISrcModelName=[]}
      mask prompts: webBlockType "WebBlock Type"; HMISrcModelName "Source Model"
      mask Help: helpview([docroot '/mapfiles/simulink.map'], 'hmi_lamp')
      mask Display:
      | if strcmp(get_param(bdroot(gcb),'BlockDiagramType'), 'library')
      |     image([(matlabroot) '/toolbox/simulink/hmi/icons/Lamp.png']);
      | end
  Lamp161 : Subsystem  DialogController=hmiCreateDDGDialog  mask(MWDashboardBlock){webBlockId=d978929e-d8a2-4db8-aeb0-36868c4d66f9, webBlockType=lamp, ShowInLibBrowser=on, ShowInitialText=on, HMISrcModelName=[]}
      mask prompts: webBlockType "WebBlock Type"; HMISrcModelName "Source Model"
      mask Help: helpview([docroot '/mapfiles/simulink.map'], 'hmi_lamp')
      mask Display:
      | if strcmp(get_param(bdroot(gcb),'BlockDiagramType'), 'library')
      |     image([(matlabroot) '/toolbox/simulink/hmi/icons/Lamp.png']);
      | end
  Lamp162 : Subsystem  DialogController=hmiCreateDDGDialog  mask(MWDashboardBlock){webBlockId=cbd10bcb-a031-4fd1-ae71-35e3b8ce37a4, webBlockType=lamp, ShowInLibBrowser=on, ShowInitialText=on, HMISrcModelName=[]}
      mask prompts: webBlockType "WebBlock Type"; HMISrcModelName "Source Model"
      mask Help: helpview([docroot '/mapfiles/simulink.map'], 'hmi_lamp')
      mask Display:
      | if strcmp(get_param(bdroot(gcb),'BlockDiagramType'), 'library')
      |     image([(matlabroot) '/toolbox/simulink/hmi/icons/Lamp.png']);
      | end
  Lamp163 : Subsystem  DialogController=hmiCreateDDGDialog  mask(MWDashboardBlock){webBlockId=c71f9eab-e84b-41df-90ee-bdab4fc5f955, webBlockType=lamp, ShowInLibBrowser=on, ShowInitialText=on, HMISrcModelName=[]}
      mask prompts: webBlockType "WebBlock Type"; HMISrcModelName "Source Model"
      mask Help: helpview([docroot '/mapfiles/simulink.map'], 'hmi_lamp')
      mask Display:
      | if strcmp(get_param(bdroot(gcb),'BlockDiagramType'), 'library')
      |     image([(matlabroot) '/toolbox/simulink/hmi/icons/Lamp.png']);
      | end
  Lamp164 : Subsystem  DialogController=hmiCreateDDGDialog  mask(MWDashboardBlock){webBlockId=1b0ed1c8-aaa5-4c0b-a202-42e16487c0de, webBlockType=lamp, ShowInLibBrowser=on, ShowInitialText=on, HMISrcModelName=[]}
      mask prompts: webBlockType "WebBlock Type"; HMISrcModelName "Source Model"
      mask Help: helpview([docroot '/mapfiles/simulink.map'], 'hmi_lamp')
      mask Display:
      | if strcmp(get_param(bdroot(gcb),'BlockDiagramType'), 'library')
      |     image([(matlabroot) '/toolbox/simulink/hmi/icons/Lamp.png']);
      | end
  Lamp165 : Subsystem  DialogController=hmiCreateDDGDialog  mask(MWDashboardBlock){webBlockId=620c51ba-7b2e-4cf7-a9db-b8e1859cb706, webBlockType=lamp, ShowInLibBrowser=on, ShowInitialText=on, HMISrcModelName=[]}
      mask prompts: webBlockType "WebBlock Type"; HMISrcModelName "Source Model"
      mask Help: helpview([docroot '/mapfiles/simulink.map'], 'hmi_lamp')
      mask Display:
      | if strcmp(get_param(bdroot(gcb),'BlockDiagramType'), 'library')
      |     image([(matlabroot) '/toolbox/simulink/hmi/icons/Lamp.png']);
      | end
  Lamp166 : Subsystem  DialogController=hmiCreateDDGDialog  mask(MWDashboardBlock){webBlockId=1917fc47-9944-41ac-8d9e-b18d83781e2e, webBlockType=lamp, ShowInLibBrowser=on, ShowInitialText=on, HMISrcModelName=[]}
      mask prompts: webBlockType "WebBlock Type"; HMISrcModelName "Source Model"
      mask Help: helpview([docroot '/mapfiles/simulink.map'], 'hmi_lamp')
      mask Display:
      | if strcmp(get_param(bdroot(gcb),'BlockDiagramType'), 'library')
      |     image([(matlabroot) '/toolbox/simulink/hmi/icons/Lamp.png']);
      | end
  Lamp167 : Subsystem  DialogController=hmiCreateDDGDialog  mask(MWDashboardBlock){webBlockId=6b527bb3-cc9d-40e5-8201-929d4d7f1832, webBlockType=lamp, ShowInLibBrowser=on, ShowInitialText=on, HMISrcModelName=[]}
      mask prompts: webBlockType "WebBlock Type"; HMISrcModelName "Source Model"
      mask Help: helpview([docroot '/mapfiles/simulink.map'], 'hmi_lamp')
      mask Display:
      | if strcmp(get_param(bdroot(gcb),'BlockDiagramType'), 'library')
      |     image([(matlabroot) '/toolbox/simulink/hmi/icons/Lamp.png']);
      | end
  Lamp168 : Subsystem  DialogController=hmiCreateDDGDialog  mask(MWDashboardBlock){webBlockId=ca0b2e5b-c405-44e4-9ed1-2b18b246efed, webBlockType=lamp, ShowInLibBrowser=on, ShowInitialText=on, HMISrcModelName=[]}
      mask prompts: webBlockType "WebBlock Type"; HMISrcModelName "Source Model"
      mask Help: helpview([docroot '/mapfiles/simulink.map'], 'hmi_lamp')
      mask Display:
      | if strcmp(get_param(bdroot(gcb),'BlockDiagramType'), 'library')
      |     image([(matlabroot) '/toolbox/simulink/hmi/icons/Lamp.png']);
      | end
  Lamp169 : Subsystem  DialogController=hmiCreateDDGDialog  mask(MWDashboardBlock){webBlockId=a8728b38-79da-4586-a2a3-8947767ce0b7, webBlockType=lamp, ShowInLibBrowser=on, ShowInitialText=on, HMISrcModelName=[]}
      mask prompts: webBlockType "WebBlock Type"; HMISrcModelName "Source Model"
      mask Help: helpview([docroot '/mapfiles/simulink.map'], 'hmi_lamp')
      mask Display:
      | if strcmp(get_param(bdroot(gcb),'BlockDiagramType'), 'library')
      |     image([(matlabroot) '/toolbox/simulink/hmi/icons/Lamp.png']);
      | end
  Lamp17 : Subsystem  DialogController=hmiCreateDDGDialog  mask(MWDashboardBlock){webBlockId=fd149fae-1681-4527-93a6-040f89cc14f5, webBlockType=lamp, ShowInLibBrowser=on, ShowInitialText=on, HMISrcModelName=[]}
      mask prompts: webBlockType "WebBlock Type"; HMISrcModelName "Source Model"
      mask Help: helpview([docroot '/mapfiles/simulink.map'], 'hmi_lamp')
      mask Display:
      | if strcmp(get_param(bdroot(gcb),'BlockDiagramType'), 'library')
      |     image([(matlabroot) '/toolbox/simulink/hmi/icons/Lamp.png']);
      | end
  Lamp170 : Subsystem  DialogController=hmiCreateDDGDialog  mask(MWDashboardBlock){webBlockId=4dc10ffd-34df-407e-9b18-a813d8980242, webBlockType=lamp, ShowInLibBrowser=on, ShowInitialText=on, HMISrcModelName=[]}
      mask prompts: webBlockType "WebBlock Type"; HMISrcModelName "Source Model"
      mask Help: helpview([docroot '/mapfiles/simulink.map'], 'hmi_lamp')
      mask Display:
      | if strcmp(get_param(bdroot(gcb),'BlockDiagramType'), 'library')
      |     image([(matlabroot) '/toolbox/simulink/hmi/icons/Lamp.png']);
      | end
  Lamp171 : Subsystem  DialogController=hmiCreateDDGDialog  mask(MWDashboardBlock){webBlockId=2277c9d5-b9d4-4193-8d81-3567d5b85eb1, webBlockType=lamp, ShowInLibBrowser=on, ShowInitialText=on, HMISrcModelName=[]}
      mask prompts: webBlockType "WebBlock Type"; HMISrcModelName "Source Model"
      mask Help: helpview([docroot '/mapfiles/simulink.map'], 'hmi_lamp')
      mask Display:
      | if strcmp(get_param(bdroot(gcb),'BlockDiagramType'), 'library')
      |     image([(matlabroot) '/toolbox/simulink/hmi/icons/Lamp.png']);
      | end
  Lamp172 : Subsystem  DialogController=hmiCreateDDGDialog  mask(MWDashboardBlock){webBlockId=78ba09b3-d748-4a35-886e-d845717b2eb7, webBlockType=lamp, ShowInLibBrowser=on, ShowInitialText=on, HMISrcModelName=[]}
      mask prompts: webBlockType "WebBlock Type"; HMISrcModelName "Source Model"
      mask Help: helpview([docroot '/mapfiles/simulink.map'], 'hmi_lamp')
      mask Display:
      | if strcmp(get_param(bdroot(gcb),'BlockDiagramType'), 'library')
      |     image([(matlabroot) '/toolbox/simulink/hmi/icons/Lamp.png']);
      | end
  Lamp173 : Subsystem  DialogController=hmiCreateDDGDialog  mask(MWDashboardBlock){webBlockId=3178a6dd-c6c2-4d14-acf0-8d1a5b0a7b04, webBlockType=lamp, ShowInLibBrowser=on, ShowInitialText=on, HMISrcModelName=[]}
      mask prompts: webBlockType "WebBlock Type"; HMISrcModelName "Source Model"
      mask Help: helpview([docroot '/mapfiles/simulink.map'], 'hmi_lamp')
      mask Display:
      | if strcmp(get_param(bdroot(gcb),'BlockDiagramType'), 'library')
      |     image([(matlabroot) '/toolbox/simulink/hmi/icons/Lamp.png']);
      | end
  Lamp174 : Subsystem  DialogController=hmiCreateDDGDialog  mask(MWDashboardBlock){webBlockId=3d74d59b-7146-4e9b-ab05-6a3aa8041d61, webBlockType=lamp, ShowInLibBrowser=on, ShowInitialText=on, HMISrcModelName=[]}
      mask prompts: webBlockType "WebBlock Type"; HMISrcModelName "Source Model"
      mask Help: helpview([docroot '/mapfiles/simulink.map'], 'hmi_lamp')
      mask Display:
      | if strcmp(get_param(bdroot(gcb),'BlockDiagramType'), 'library')
      |     image([(matlabroot) '/toolbox/simulink/hmi/icons/Lamp.png']);
      | end
  Lamp175 : Subsystem  DialogController=hmiCreateDDGDialog  mask(MWDashboardBlock){webBlockId=9e936e91-41a4-4049-acd8-534c0cf76138, webBlockType=lamp, ShowInLibBrowser=on, ShowInitialText=on, HMISrcModelName=[]}
      mask prompts: webBlockType "WebBlock Type"; HMISrcModelName "Source Model"
      mask Help: helpview([docroot '/mapfiles/simulink.map'], 'hmi_lamp')
      mask Display:
      | if strcmp(get_param(bdroot(gcb),'BlockDiagramType'), 'library')
      |     image([(matlabroot) '/toolbox/simulink/hmi/icons/Lamp.png']);
      | end
  Lamp176 : Subsystem  DialogController=hmiCreateDDGDialog  mask(MWDashboardBlock){webBlockId=5c7a1377-28bc-441e-bf8a-d4d0b50c22f0, webBlockType=lamp, ShowInLibBrowser=on, ShowInitialText=on, HMISrcModelName=[]}
      mask prompts: webBlockType "WebBlock Type"; HMISrcModelName "Source Model"
      mask Help: helpview([docroot '/mapfiles/simulink.map'], 'hmi_lamp')
      mask Display:
      | if strcmp(get_param(bdroot(gcb),'BlockDiagramType'), 'library')
      |     image([(matlabroot) '/toolbox/simulink/hmi/icons/Lamp.png']);
      | end
  Lamp177 : Subsystem  DialogController=hmiCreateDDGDialog  mask(MWDashboardBlock){webBlockId=11ac63d7-eb90-4cb0-a267-f2c869149d84, webBlockType=lamp, ShowInLibBrowser=on, ShowInitialText=on, HMISrcModelName=[]}
      mask prompts: webBlockType "WebBlock Type"; HMISrcModelName "Source Model"
      mask Help: helpview([docroot '/mapfiles/simulink.map'], 'hmi_lamp')
      mask Display:
      | if strcmp(get_param(bdroot(gcb),'BlockDiagramType'), 'library')
      |     image([(matlabroot) '/toolbox/simulink/hmi/icons/Lamp.png']);
      | end
  Lamp178 : Subsystem  DialogController=hmiCreateDDGDialog  mask(MWDashboardBlock){webBlockId=1ccf8047-cdef-4e36-8a21-17b06839429f, webBlockType=lamp, ShowInLibBrowser=on, ShowInitialText=on, HMISrcModelName=[]}
      mask prompts: webBlockType "WebBlock Type"; HMISrcModelName "Source Model"
      mask Help: helpview([docroot '/mapfiles/simulink.map'], 'hmi_lamp')
      mask Display:
      | if strcmp(get_param(bdroot(gcb),'BlockDiagramType'), 'library')
      |     image([(matlabroot) '/toolbox/simulink/hmi/icons/Lamp.png']);
      | end
  Lamp179 : Subsystem  DialogController=hmiCreateDDGDialog  mask(MWDashboardBlock){webBlockId=fe862bea-ba0b-4f41-86a9-a0b3926481da, webBlockType=lamp, ShowInLibBrowser=on, ShowInitialText=on, HMISrcModelName=[]}
      mask prompts: webBlockType "WebBlock Type"; HMISrcModelName "Source Model"
      mask Help: helpview([docroot '/mapfiles/simulink.map'], 'hmi_lamp')
      mask Display:
      | if strcmp(get_param(bdroot(gcb),'BlockDiagramType'), 'library')
      |     image([(matlabroot) '/toolbox/simulink/hmi/icons/Lamp.png']);
      | end
  Lamp18 : Subsystem  DialogController=hmiCreateDDGDialog  mask(MWDashboardBlock){webBlockId=578d50d4-b1ca-441f-a725-e8ae220ff61c, webBlockType=lamp, ShowInLibBrowser=on, ShowInitialText=on, HMISrcModelName=[]}
      mask prompts: webBlockType "WebBlock Type"; HMISrcModelName "Source Model"
      mask Help: helpview([docroot '/mapfiles/simulink.map'], 'hmi_lamp')
      mask Display:
      | if strcmp(get_param(bdroot(gcb),'BlockDiagramType'), 'library')
      |     image([(matlabroot) '/toolbox/simulink/hmi/icons/Lamp.png']);
      | end
  Lamp180 : Subsystem  DialogController=hmiCreateDDGDialog  mask(MWDashboardBlock){webBlockId=edf824f8-a7e3-43c0-9277-b4e793c8aae3, webBlockType=lamp, ShowInLibBrowser=on, ShowInitialText=on, HMISrcModelName=[]}
      mask prompts: webBlockType "WebBlock Type"; HMISrcModelName "Source Model"
      mask Help: helpview([docroot '/mapfiles/simulink.map'], 'hmi_lamp')
      mask Display:
      | if strcmp(get_param(bdroot(gcb),'BlockDiagramType'), 'library')
      |     image([(matlabroot) '/toolbox/simulink/hmi/icons/Lamp.png']);
      | end
  Lamp181 : Subsystem  DialogController=hmiCreateDDGDialog  mask(MWDashboardBlock){webBlockId=457a6c8d-adaf-4186-ae45-8befa26723d3, webBlockType=lamp, ShowInLibBrowser=on, ShowInitialText=on, HMISrcModelName=[]}
      mask prompts: webBlockType "WebBlock Type"; HMISrcModelName "Source Model"
      mask Help: helpview([docroot '/mapfiles/simulink.map'], 'hmi_lamp')
      mask Display:
      | if strcmp(get_param(bdroot(gcb),'BlockDiagramType'), 'library')
      |     image([(matlabroot) '/toolbox/simulink/hmi/icons/Lamp.png']);
      | end
  Lamp182 : Subsystem  DialogController=hmiCreateDDGDialog  mask(MWDashboardBlock){webBlockId=fb475414-b146-4484-8113-68f8b4285f2f, webBlockType=lamp, ShowInLibBrowser=on, ShowInitialText=on, HMISrcModelName=[]}
      mask prompts: webBlockType "WebBlock Type"; HMISrcModelName "Source Model"
      mask Help: helpview([docroot '/mapfiles/simulink.map'], 'hmi_lamp')
      mask Display:
      | if strcmp(get_param(bdroot(gcb),'BlockDiagramType'), 'library')
      |     image([(matlabroot) '/toolbox/simulink/hmi/icons/Lamp.png']);
      | end
  Lamp183 : Subsystem  DialogController=hmiCreateDDGDialog  mask(MWDashboardBlock){webBlockId=31daa029-828e-4985-9d06-0eb8b530fc8e, webBlockType=lamp, ShowInLibBrowser=on, ShowInitialText=on, HMISrcModelName=[]}
      mask prompts: webBlockType "WebBlock Type"; HMISrcModelName "Source Model"
      mask Help: helpview([docroot '/mapfiles/simulink.map'], 'hmi_lamp')
      mask Display:
      | if strcmp(get_param(bdroot(gcb),'BlockDiagramType'), 'library')
      |     image([(matlabroot) '/toolbox/simulink/hmi/icons/Lamp.png']);
      | end
  Lamp184 : Subsystem  DialogController=hmiCreateDDGDialog  mask(MWDashboardBlock){webBlockId=ecad05a4-a7ae-4249-a486-94dbac563c79, webBlockType=lamp, ShowInLibBrowser=on, ShowInitialText=on, HMISrcModelName=[]}
      mask prompts: webBlockType "WebBlock Type"; HMISrcModelName "Source Model"
      mask Help: helpview([docroot '/mapfiles/simulink.map'], 'hmi_lamp')
      mask Display:
      | if strcmp(get_param(bdroot(gcb),'BlockDiagramType'), 'library')
      |     image([(matlabroot) '/toolbox/simulink/hmi/icons/Lamp.png']);
      | end
  Lamp185 : Subsystem  DialogController=hmiCreateDDGDialog  mask(MWDashboardBlock){webBlockId=d8e6c8bc-5b86-40b0-8396-fb5089cc3107, webBlockType=lamp, ShowInLibBrowser=on, ShowInitialText=on, HMISrcModelName=[]}
      mask prompts: webBlockType "WebBlock Type"; HMISrcModelName "Source Model"
      mask Help: helpview([docroot '/mapfiles/simulink.map'], 'hmi_lamp')
      mask Display:
      | if strcmp(get_param(bdroot(gcb),'BlockDiagramType'), 'library')
      |     image([(matlabroot) '/toolbox/simulink/hmi/icons/Lamp.png']);
      | end
  Lamp186 : Subsystem  DialogController=hmiCreateDDGDialog  mask(MWDashboardBlock){webBlockId=4007698d-26f1-4f3b-bc2b-093afd0e962c, webBlockType=lamp, ShowInLibBrowser=on, ShowInitialText=on, HMISrcModelName=[]}
      mask prompts: webBlockType "WebBlock Type"; HMISrcModelName "Source Model"
      mask Help: helpview([docroot '/mapfiles/simulink.map'], 'hmi_lamp')
      mask Display:
      | if strcmp(get_param(bdroot(gcb),'BlockDiagramType'), 'library')
      |     image([(matlabroot) '/toolbox/simulink/hmi/icons/Lamp.png']);
      | end
  Lamp187 : Subsystem  DialogController=hmiCreateDDGDialog  mask(MWDashboardBlock){webBlockId=1974d0b5-35b0-4ed8-8ddb-ea3bd9d5c405, webBlockType=lamp, ShowInLibBrowser=on, ShowInitialText=on, HMISrcModelName=[]}
      mask prompts: webBlockType "WebBlock Type"; HMISrcModelName "Source Model"
      mask Help: helpview([docroot '/mapfiles/simulink.map'], 'hmi_lamp')
      mask Display:
      | if strcmp(get_param(bdroot(gcb),'BlockDiagramType'), 'library')
      |     image([(matlabroot) '/toolbox/simulink/hmi/icons/Lamp.png']);
      | end
  Lamp188 : Subsystem  DialogController=hmiCreateDDGDialog  mask(MWDashboardBlock){webBlockId=f320a457-dbce-4b35-8849-1999327e42cb, webBlockType=lamp, ShowInLibBrowser=on, ShowInitialText=on, HMISrcModelName=[]}
      mask prompts: webBlockType "WebBlock Type"; HMISrcModelName "Source Model"
      mask Help: helpview([docroot '/mapfiles/simulink.map'], 'hmi_lamp')
      mask Display:
      | if strcmp(get_param(bdroot(gcb),'BlockDiagramType'), 'library')
      |     image([(matlabroot) '/toolbox/simulink/hmi/icons/Lamp.png']);
      | end
  Lamp189 : Subsystem  DialogController=hmiCreateDDGDialog  mask(MWDashboardBlock){webBlockId=37d5035d-398b-4cf9-85f7-b8569ce417c9, webBlockType=lamp, ShowInLibBrowser=on, ShowInitialText=on, HMISrcModelName=[]}
      mask prompts: webBlockType "WebBlock Type"; HMISrcModelName "Source Model"
      mask Help: helpview([docroot '/mapfiles/simulink.map'], 'hmi_lamp')
      mask Display:
      | if strcmp(get_param(bdroot(gcb),'BlockDiagramType'), 'library')
      |     image([(matlabroot) '/toolbox/simulink/hmi/icons/Lamp.png']);
      | end
  Lamp19 : Subsystem  DialogController=hmiCreateDDGDialog  mask(MWDashboardBlock){webBlockId=8675453f-3a9f-4b19-8f2d-bcd149e3d70c, webBlockType=lamp, ShowInLibBrowser=on, ShowInitialText=on, HMISrcModelName=[]}
      mask prompts: webBlockType "WebBlock Type"; HMISrcModelName "Source Model"
      mask Help: helpview([docroot '/mapfiles/simulink.map'], 'hmi_lamp')
      mask Display:
      | if strcmp(get_param(bdroot(gcb),'BlockDiagramType'), 'library')
      |     image([(matlabroot) '/toolbox/simulink/hmi/icons/Lamp.png']);
      | end
  Lamp190 : Subsystem  DialogController=hmiCreateDDGDialog  mask(MWDashboardBlock){webBlockId=1e7f5f0a-8a97-4007-8b88-0f2a06eb1bc6, webBlockType=lamp, ShowInLibBrowser=on, ShowInitialText=on, HMISrcModelName=[]}
      mask prompts: webBlockType "WebBlock Type"; HMISrcModelName "Source Model"
      mask Help: helpview([docroot '/mapfiles/simulink.map'], 'hmi_lamp')
      mask Display:
      | if strcmp(get_param(bdroot(gcb),'BlockDiagramType'), 'library')
      |     image([(matlabroot) '/toolbox/simulink/hmi/icons/Lamp.png']);
      | end
  Lamp191 : Subsystem  DialogController=hmiCreateDDGDialog  mask(MWDashboardBlock){webBlockId=d42ecdd5-c19a-4dad-b775-3f0bb4c70156, webBlockType=lamp, ShowInLibBrowser=on, ShowInitialText=on, HMISrcModelName=[]}
      mask prompts: webBlockType "WebBlock Type"; HMISrcModelName "Source Model"
      mask Help: helpview([docroot '/mapfiles/simulink.map'], 'hmi_lamp')
      mask Display:
      | if strcmp(get_param(bdroot(gcb),'BlockDiagramType'), 'library')
      |     image([(matlabroot) '/toolbox/simulink/hmi/icons/Lamp.png']);
      | end
  Lamp192 : Subsystem  DialogController=hmiCreateDDGDialog  mask(MWDashboardBlock){webBlockId=b4ebe065-9f3c-4e0e-a20e-42188a50d346, webBlockType=lamp, ShowInLibBrowser=on, ShowInitialText=on, HMISrcModelName=[]}
      mask prompts: webBlockType "WebBlock Type"; HMISrcModelName "Source Model"
      mask Help: helpview([docroot '/mapfiles/simulink.map'], 'hmi_lamp')
      mask Display:
      | if strcmp(get_param(bdroot(gcb),'BlockDiagramType'), 'library')
      |     image([(matlabroot) '/toolbox/simulink/hmi/icons/Lamp.png']);
      | end
  Lamp193 : Subsystem  DialogController=hmiCreateDDGDialog  mask(MWDashboardBlock){webBlockId=a646259e-e68a-4174-a18a-ee51c5656218, webBlockType=lamp, ShowInLibBrowser=on, ShowInitialText=on, HMISrcModelName=[]}
      mask prompts: webBlockType "WebBlock Type"; HMISrcModelName "Source Model"
      mask Help: helpview([docroot '/mapfiles/simulink.map'], 'hmi_lamp')
      mask Display:
      | if strcmp(get_param(bdroot(gcb),'BlockDiagramType'), 'library')
      |     image([(matlabroot) '/toolbox/simulink/hmi/icons/Lamp.png']);
      | end
  Lamp194 : Subsystem  DialogController=hmiCreateDDGDialog  mask(MWDashboardBlock){webBlockId=a2833e00-c9b8-462e-bdea-0f712142d6e9, webBlockType=lamp, ShowInLibBrowser=on, ShowInitialText=on, HMISrcModelName=[]}
      mask prompts: webBlockType "WebBlock Type"; HMISrcModelName "Source Model"
      mask Help: helpview([docroot '/mapfiles/simulink.map'], 'hmi_lamp')
      mask Display:
      | if strcmp(get_param(bdroot(gcb),'BlockDiagramType'), 'library')
      |     image([(matlabroot) '/toolbox/simulink/hmi/icons/Lamp.png']);
      | end
  Lamp195 : Subsystem  DialogController=hmiCreateDDGDialog  mask(MWDashboardBlock){webBlockId=ef4f1330-6665-410d-a56b-54762f2d9036, webBlockType=lamp, ShowInLibBrowser=on, ShowInitialText=on, HMISrcModelName=[]}
      mask prompts: webBlockType "WebBlock Type"; HMISrcModelName "Source Model"
      mask Help: helpview([docroot '/mapfiles/simulink.map'], 'hmi_lamp')
      mask Display:
      | if strcmp(get_param(bdroot(gcb),'BlockDiagramType'), 'library')
      |     image([(matlabroot) '/toolbox/simulink/hmi/icons/Lamp.png']);
      | end
  Lamp196 : Subsystem  DialogController=hmiCreateDDGDialog  mask(MWDashboardBlock){webBlockId=baa20663-d2b4-42f7-b061-0389350871be, webBlockType=lamp, ShowInLibBrowser=on, ShowInitialText=on, HMISrcModelName=[]}
      mask prompts: webBlockType "WebBlock Type"; HMISrcModelName "Source Model"
      mask Help: helpview([docroot '/mapfiles/simulink.map'], 'hmi_lamp')
      mask Display:
      | if strcmp(get_param(bdroot(gcb),'BlockDiagramType'), 'library')
      |     image([(matlabroot) '/toolbox/simulink/hmi/icons/Lamp.png']);
      | end
  Lamp197 : Subsystem  DialogController=hmiCreateDDGDialog  mask(MWDashboardBlock){webBlockId=c3ca63c9-1ed3-45be-8b11-5490da322155, webBlockType=lamp, ShowInLibBrowser=on, ShowInitialText=on, HMISrcModelName=[]}
      mask prompts: webBlockType "WebBlock Type"; HMISrcModelName "Source Model"
      mask Help: helpview([docroot '/mapfiles/simulink.map'], 'hmi_lamp')
      mask Display:
      | if strcmp(get_param(bdroot(gcb),'BlockDiagramType'), 'library')
      |     image([(matlabroot) '/toolbox/simulink/hmi/icons/Lamp.png']);
      | end
  Lamp198 : Subsystem  DialogController=hmiCreateDDGDialog  mask(MWDashboardBlock){webBlockId=5a6ae0b6-460e-45df-96c4-dd3af88c4bfb, webBlockType=lamp, ShowInLibBrowser=on, ShowInitialText=on, HMISrcModelName=[]}
      mask prompts: webBlockType "WebBlock Type"; HMISrcModelName "Source Model"
      mask Help: helpview([docroot '/mapfiles/simulink.map'], 'hmi_lamp')
      mask Display:
      | if strcmp(get_param(bdroot(gcb),'BlockDiagramType'), 'library')
      |     image([(matlabroot) '/toolbox/simulink/hmi/icons/Lamp.png']);
      | end
  Lamp199 : Subsystem  DialogController=hmiCreateDDGDialog  mask(MWDashboardBlock){webBlockId=5ad091db-045c-4a72-8d85-6c8cc82b129d, webBlockType=lamp, ShowInLibBrowser=on, ShowInitialText=on, HMISrcModelName=[]}
      mask prompts: webBlockType "WebBlock Type"; HMISrcModelName "Source Model"
      mask Help: helpview([docroot '/mapfiles/simulink.map'], 'hmi_lamp')
      mask Display:
      | if strcmp(get_param(bdroot(gcb),'BlockDiagramType'), 'library')
      |     image([(matlabroot) '/toolbox/simulink/hmi/icons/Lamp.png']);
      | end
  Lamp2 : Subsystem  DialogController=hmiCreateDDGDialog  mask(MWDashboardBlock){webBlockId=2a0feb0f-7815-4e75-a54c-c124100acebb, webBlockType=lamp, ShowInLibBrowser=on, ShowInitialText=on, HMISrcModelName=[]}
      mask prompts: webBlockType "WebBlock Type"; HMISrcModelName "Source Model"
      mask Help: helpview([docroot '/mapfiles/simulink.map'], 'hmi_lamp')
      mask Display:
      | if strcmp(get_param(bdroot(gcb),'BlockDiagramType'), 'library')
      |     image([(matlabroot) '/toolbox/simulink/hmi/icons/Lamp.png']);
      | end
  Lamp20 : Subsystem  DialogController=hmiCreateDDGDialog  mask(MWDashboardBlock){webBlockId=524ba15c-be26-4050-b236-7b01adf0c405, webBlockType=lamp, ShowInLibBrowser=on, ShowInitialText=on, HMISrcModelName=[]}
      mask prompts: webBlockType "WebBlock Type"; HMISrcModelName "Source Model"
      mask Help: helpview([docroot '/mapfiles/simulink.map'], 'hmi_lamp')
      mask Display:
      | if strcmp(get_param(bdroot(gcb),'BlockDiagramType'), 'library')
      |     image([(matlabroot) '/toolbox/simulink/hmi/icons/Lamp.png']);
      | end
  Lamp200 : Subsystem  DialogController=hmiCreateDDGDialog  mask(MWDashboardBlock){webBlockId=5ac6faec-1839-48f1-8b9b-597b35c6163d, webBlockType=lamp, ShowInLibBrowser=on, ShowInitialText=on, HMISrcModelName=[]}
      mask prompts: webBlockType "WebBlock Type"; HMISrcModelName "Source Model"
      mask Help: helpview([docroot '/mapfiles/simulink.map'], 'hmi_lamp')
      mask Display:
      | if strcmp(get_param(bdroot(gcb),'BlockDiagramType'), 'library')
      |     image([(matlabroot) '/toolbox/simulink/hmi/icons/Lamp.png']);
      | end
  Lamp201 : Subsystem  DialogController=hmiCreateDDGDialog  mask(MWDashboardBlock){webBlockId=073dfa11-fd1a-49ee-b3a9-877d9fec153e, webBlockType=lamp, ShowInLibBrowser=on, ShowInitialText=on, HMISrcModelName=[]}
      mask prompts: webBlockType "WebBlock Type"; HMISrcModelName "Source Model"
      mask Help: helpview([docroot '/mapfiles/simulink.map'], 'hmi_lamp')
      mask Display:
      | if strcmp(get_param(bdroot(gcb),'BlockDiagramType'), 'library')
      |     image([(matlabroot) '/toolbox/simulink/hmi/icons/Lamp.png']);
      | end
  Lamp202 : Subsystem  DialogController=hmiCreateDDGDialog  mask(MWDashboardBlock){webBlockId=e0b4136d-6999-492a-8ebb-63c9d673511f, webBlockType=lamp, ShowInLibBrowser=on, ShowInitialText=on, HMISrcModelName=[]}
      mask prompts: webBlockType "WebBlock Type"; HMISrcModelName "Source Model"
      mask Help: helpview([docroot '/mapfiles/simulink.map'], 'hmi_lamp')
      mask Display:
      | if strcmp(get_param(bdroot(gcb),'BlockDiagramType'), 'library')
      |     image([(matlabroot) '/toolbox/simulink/hmi/icons/Lamp.png']);
      | end
  Lamp203 : Subsystem  DialogController=hmiCreateDDGDialog  mask(MWDashboardBlock){webBlockId=9df63901-5e59-476a-917f-a5e59ffbf1a0, webBlockType=lamp, ShowInLibBrowser=on, ShowInitialText=on, HMISrcModelName=[]}
      mask prompts: webBlockType "WebBlock Type"; HMISrcModelName "Source Model"
      mask Help: helpview([docroot '/mapfiles/simulink.map'], 'hmi_lamp')
      mask Display:
      | if strcmp(get_param(bdroot(gcb),'BlockDiagramType'), 'library')
      |     image([(matlabroot) '/toolbox/simulink/hmi/icons/Lamp.png']);
      | end
  Lamp204 : Subsystem  DialogController=hmiCreateDDGDialog  mask(MWDashboardBlock){webBlockId=99f7c8bc-1cc1-4766-a52a-7f5d3c197f07, webBlockType=lamp, ShowInLibBrowser=on, ShowInitialText=on, HMISrcModelName=[]}
      mask prompts: webBlockType "WebBlock Type"; HMISrcModelName "Source Model"
      mask Help: helpview([docroot '/mapfiles/simulink.map'], 'hmi_lamp')
      mask Display:
      | if strcmp(get_param(bdroot(gcb),'BlockDiagramType'), 'library')
      |     image([(matlabroot) '/toolbox/simulink/hmi/icons/Lamp.png']);
      | end
  Lamp205 : Subsystem  DialogController=hmiCreateDDGDialog  mask(MWDashboardBlock){webBlockId=850e8768-4397-4434-b57c-b485c2547c46, webBlockType=lamp, ShowInLibBrowser=on, ShowInitialText=on, HMISrcModelName=[]}
      mask prompts: webBlockType "WebBlock Type"; HMISrcModelName "Source Model"
      mask Help: helpview([docroot '/mapfiles/simulink.map'], 'hmi_lamp')
      mask Display:
      | if strcmp(get_param(bdroot(gcb),'BlockDiagramType'), 'library')
      |     image([(matlabroot) '/toolbox/simulink/hmi/icons/Lamp.png']);
      | end
  Lamp206 : Subsystem  DialogController=hmiCreateDDGDialog  mask(MWDashboardBlock){webBlockId=7ed3901b-7c8c-4d95-ae62-8f22a9025245, webBlockType=lamp, ShowInLibBrowser=on, ShowInitialText=on, HMISrcModelName=[]}
      mask prompts: webBlockType "WebBlock Type"; HMISrcModelName "Source Model"
      mask Help: helpview([docroot '/mapfiles/simulink.map'], 'hmi_lamp')
      mask Display:
      | if strcmp(get_param(bdroot(gcb),'BlockDiagramType'), 'library')
      |     image([(matlabroot) '/toolbox/simulink/hmi/icons/Lamp.png']);
      | end
  Lamp207 : Subsystem  DialogController=hmiCreateDDGDialog  mask(MWDashboardBlock){webBlockId=c2ea2193-146a-47c1-bd5f-c3c63ac2329c, webBlockType=lamp, ShowInLibBrowser=on, ShowInitialText=on, HMISrcModelName=[]}
      mask prompts: webBlockType "WebBlock Type"; HMISrcModelName "Source Model"
      mask Help: helpview([docroot '/mapfiles/simulink.map'], 'hmi_lamp')
      mask Display:
      | if strcmp(get_param(bdroot(gcb),'BlockDiagramType'), 'library')
      |     image([(matlabroot) '/toolbox/simulink/hmi/icons/Lamp.png']);
      | end
  Lamp208 : Subsystem  DialogController=hmiCreateDDGDialog  mask(MWDashboardBlock){webBlockId=c2aad158-2a48-414a-a5ab-20b62812acd9, webBlockType=lamp, ShowInLibBrowser=on, ShowInitialText=on, HMISrcModelName=[]}
      mask prompts: webBlockType "WebBlock Type"; HMISrcModelName "Source Model"
      mask Help: helpview([docroot '/mapfiles/simulink.map'], 'hmi_lamp')
      mask Display:
      | if strcmp(get_param(bdroot(gcb),'BlockDiagramType'), 'library')
      |     image([(matlabroot) '/toolbox/simulink/hmi/icons/Lamp.png']);
      | end
  Lamp209 : Subsystem  DialogController=hmiCreateDDGDialog  mask(MWDashboardBlock){webBlockId=b6bf220d-6463-45fb-9c47-1568c6ef1c61, webBlockType=lamp, ShowInLibBrowser=on, ShowInitialText=on, HMISrcModelName=[]}
      mask prompts: webBlockType "WebBlock Type"; HMISrcModelName "Source Model"
      mask Help: helpview([docroot '/mapfiles/simulink.map'], 'hmi_lamp')
      mask Display:
      | if strcmp(get_param(bdroot(gcb),'BlockDiagramType'), 'library')
      |     image([(matlabroot) '/toolbox/simulink/hmi/icons/Lamp.png']);
      | end
  Lamp21 : Subsystem  DialogController=hmiCreateDDGDialog  mask(MWDashboardBlock){webBlockId=49b5e6f7-d9bf-4305-9cda-42ad87644046, webBlockType=lamp, ShowInLibBrowser=on, ShowInitialText=on, HMISrcModelName=[]}
      mask prompts: webBlockType "WebBlock Type"; HMISrcModelName "Source Model"
      mask Help: helpview([docroot '/mapfiles/simulink.map'], 'hmi_lamp')
      mask Display:
      | if strcmp(get_param(bdroot(gcb),'BlockDiagramType'), 'library')
      |     image([(matlabroot) '/toolbox/simulink/hmi/icons/Lamp.png']);
      | end
  Lamp210 : Subsystem  DialogController=hmiCreateDDGDialog  mask(MWDashboardBlock){webBlockId=8abbf899-44f6-40e9-9652-9d71a2baee31, webBlockType=lamp, ShowInLibBrowser=on, ShowInitialText=on, HMISrcModelName=[]}
      mask prompts: webBlockType "WebBlock Type"; HMISrcModelName "Source Model"
      mask Help: helpview([docroot '/mapfiles/simulink.map'], 'hmi_lamp')
      mask Display:
      | if strcmp(get_param(bdroot(gcb),'BlockDiagramType'), 'library')
      |     image([(matlabroot) '/toolbox/simulink/hmi/icons/Lamp.png']);
      | end
  Lamp211 : Subsystem  DialogController=hmiCreateDDGDialog  mask(MWDashboardBlock){webBlockId=5841e3e3-0b79-4ddb-ab6c-396db476227d, webBlockType=lamp, ShowInLibBrowser=on, ShowInitialText=on, HMISrcModelName=[]}
      mask prompts: webBlockType "WebBlock Type"; HMISrcModelName "Source Model"
      mask Help: helpview([docroot '/mapfiles/simulink.map'], 'hmi_lamp')
      mask Display:
      | if strcmp(get_param(bdroot(gcb),'BlockDiagramType'), 'library')
      |     image([(matlabroot) '/toolbox/simulink/hmi/icons/Lamp.png']);
      | end
  Lamp212 : Subsystem  DialogController=hmiCreateDDGDialog  mask(MWDashboardBlock){webBlockId=b278f8e6-8d59-40f0-ba75-6e92164c37fe, webBlockType=lamp, ShowInLibBrowser=on, ShowInitialText=on, HMISrcModelName=[]}
      mask prompts: webBlockType "WebBlock Type"; HMISrcModelName "Source Model"
      mask Help: helpview([docroot '/mapfiles/simulink.map'], 'hmi_lamp')
      mask Display:
      | if strcmp(get_param(bdroot(gcb),'BlockDiagramType'), 'library')
      |     image([(matlabroot) '/toolbox/simulink/hmi/icons/Lamp.png']);
      | end
  Lamp213 : Subsystem  DialogController=hmiCreateDDGDialog  mask(MWDashboardBlock){webBlockId=0f1542e3-9d99-4b00-8893-0073668dfd4e, webBlockType=lamp, ShowInLibBrowser=on, ShowInitialText=on, HMISrcModelName=[]}
      mask prompts: webBlockType "WebBlock Type"; HMISrcModelName "Source Model"
      mask Help: helpview([docroot '/mapfiles/simulink.map'], 'hmi_lamp')
      mask Display:
      | if strcmp(get_param(bdroot(gcb),'BlockDiagramType'), 'library')
      |     image([(matlabroot) '/toolbox/simulink/hmi/icons/Lamp.png']);
      | end
  Lamp214 : Subsystem  DialogController=hmiCreateDDGDialog  mask(MWDashboardBlock){webBlockId=be520d2f-66d6-46a7-9631-d4481e373f0f, webBlockType=lamp, ShowInLibBrowser=on, ShowInitialText=on, HMISrcModelName=[]}
      mask prompts: webBlockType "WebBlock Type"; HMISrcModelName "Source Model"
      mask Help: helpview([docroot '/mapfiles/simulink.map'], 'hmi_lamp')
      mask Display:
      | if strcmp(get_param(bdroot(gcb),'BlockDiagramType'), 'library')
      |     image([(matlabroot) '/toolbox/simulink/hmi/icons/Lamp.png']);
      | end
  Lamp215 : Subsystem  DialogController=hmiCreateDDGDialog  mask(MWDashboardBlock){webBlockId=6ef354da-5284-40ae-9168-a0aeaa86a34e, webBlockType=lamp, ShowInLibBrowser=on, ShowInitialText=on, HMISrcModelName=[]}
      mask prompts: webBlockType "WebBlock Type"; HMISrcModelName "Source Model"
      mask Help: helpview([docroot '/mapfiles/simulink.map'], 'hmi_lamp')
      mask Display:
      | if strcmp(get_param(bdroot(gcb),'BlockDiagramType'), 'library')
      |     image([(matlabroot) '/toolbox/simulink/hmi/icons/Lamp.png']);
      | end
  Lamp216 : Subsystem  DialogController=hmiCreateDDGDialog  mask(MWDashboardBlock){webBlockId=8b9d5b34-937d-4700-84dd-750a44084c01, webBlockType=lamp, ShowInLibBrowser=on, ShowInitialText=on, HMISrcModelName=[]}
      mask prompts: webBlockType "WebBlock Type"; HMISrcModelName "Source Model"
      mask Help: helpview([docroot '/mapfiles/simulink.map'], 'hmi_lamp')
      mask Display:
      | if strcmp(get_param(bdroot(gcb),'BlockDiagramType'), 'library')
      |     image([(matlabroot) '/toolbox/simulink/hmi/icons/Lamp.png']);
      | end
  Lamp217 : Subsystem  DialogController=hmiCreateDDGDialog  mask(MWDashboardBlock){webBlockId=325b186d-eefe-4f63-b119-60d25e0a8923, webBlockType=lamp, ShowInLibBrowser=on, ShowInitialText=on, HMISrcModelName=[]}
      mask prompts: webBlockType "WebBlock Type"; HMISrcModelName "Source Model"
      mask Help: helpview([docroot '/mapfiles/simulink.map'], 'hmi_lamp')
      mask Display:
      | if strcmp(get_param(bdroot(gcb),'BlockDiagramType'), 'library')
      |     image([(matlabroot) '/toolbox/simulink/hmi/icons/Lamp.png']);
      | end
  Lamp218 : Subsystem  DialogController=hmiCreateDDGDialog  mask(MWDashboardBlock){webBlockId=a9fdf443-293d-4631-bae4-ae05b8036d11, webBlockType=lamp, ShowInLibBrowser=on, ShowInitialText=on, HMISrcModelName=[]}
      mask prompts: webBlockType "WebBlock Type"; HMISrcModelName "Source Model"
      mask Help: helpview([docroot '/mapfiles/simulink.map'], 'hmi_lamp')
      mask Display:
      | if strcmp(get_param(bdroot(gcb),'BlockDiagramType'), 'library')
      |     image([(matlabroot) '/toolbox/simulink/hmi/icons/Lamp.png']);
      | end
  Lamp219 : Subsystem  DialogController=hmiCreateDDGDialog  mask(MWDashboardBlock){webBlockId=49b7d9b8-b4cc-43ab-b220-d7cec4a69c6c, webBlockType=lamp, ShowInLibBrowser=on, ShowInitialText=on, HMISrcModelName=[]}
      mask prompts: webBlockType "WebBlock Type"; HMISrcModelName "Source Model"
      mask Help: helpview([docroot '/mapfiles/simulink.map'], 'hmi_lamp')
      mask Display:
      | if strcmp(get_param(bdroot(gcb),'BlockDiagramType'), 'library')
      |     image([(matlabroot) '/toolbox/simulink/hmi/icons/Lamp.png']);
      | end
  Lamp22 : Subsystem  DialogController=hmiCreateDDGDialog  mask(MWDashboardBlock){webBlockId=396a3b8f-c424-4629-ba11-feeb444226ca, webBlockType=lamp, ShowInLibBrowser=on, ShowInitialText=on, HMISrcModelName=[]}
      mask prompts: webBlockType "WebBlock Type"; HMISrcModelName "Source Model"
      mask Help: helpview([docroot '/mapfiles/simulink.map'], 'hmi_lamp')
      mask Display:
      | if strcmp(get_param(bdroot(gcb),'BlockDiagramType'), 'library')
      |     image([(matlabroot) '/toolbox/simulink/hmi/icons/Lamp.png']);
      | end
  Lamp220 : Subsystem  DialogController=hmiCreateDDGDialog  mask(MWDashboardBlock){webBlockId=3c3b70fe-6f64-4d75-a50b-832583e4a30a, webBlockType=lamp, ShowInLibBrowser=on, ShowInitialText=on, HMISrcModelName=[]}
      mask prompts: webBlockType "WebBlock Type"; HMISrcModelName "Source Model"
      mask Help: helpview([docroot '/mapfiles/simulink.map'], 'hmi_lamp')
      mask Display:
      | if strcmp(get_param(bdroot(gcb),'BlockDiagramType'), 'library')
      |     image([(matlabroot) '/toolbox/simulink/hmi/icons/Lamp.png']);
      | end
  Lamp221 : Subsystem  DialogController=hmiCreateDDGDialog  mask(MWDashboardBlock){webBlockId=5ff5ad66-69ab-4745-b29a-6fd52a47da67, webBlockType=lamp, ShowInLibBrowser=on, ShowInitialText=on, HMISrcModelName=[]}
      mask prompts: webBlockType "WebBlock Type"; HMISrcModelName "Source Model"
      mask Help: helpview([docroot '/mapfiles/simulink.map'], 'hmi_lamp')
      mask Display:
      | if strcmp(get_param(bdroot(gcb),'BlockDiagramType'), 'library')
      |     image([(matlabroot) '/toolbox/simulink/hmi/icons/Lamp.png']);
      | end
  Lamp222 : Subsystem  DialogController=hmiCreateDDGDialog  mask(MWDashboardBlock){webBlockId=4bbe58ef-ec86-4468-8ae9-78b3e36cc35b, webBlockType=lamp, ShowInLibBrowser=on, ShowInitialText=on, HMISrcModelName=[]}
      mask prompts: webBlockType "WebBlock Type"; HMISrcModelName "Source Model"
      mask Help: helpview([docroot '/mapfiles/simulink.map'], 'hmi_lamp')
      mask Display:
      | if strcmp(get_param(bdroot(gcb),'BlockDiagramType'), 'library')
      |     image([(matlabroot) '/toolbox/simulink/hmi/icons/Lamp.png']);
      | end
  Lamp223 : Subsystem  DialogController=hmiCreateDDGDialog  mask(MWDashboardBlock){webBlockId=1c1d9e13-2cb5-42eb-9db9-4a6b33275da7, webBlockType=lamp, ShowInLibBrowser=on, ShowInitialText=on, HMISrcModelName=[]}
      mask prompts: webBlockType "WebBlock Type"; HMISrcModelName "Source Model"
      mask Help: helpview([docroot '/mapfiles/simulink.map'], 'hmi_lamp')
      mask Display:
      | if strcmp(get_param(bdroot(gcb),'BlockDiagramType'), 'library')
      |     image([(matlabroot) '/toolbox/simulink/hmi/icons/Lamp.png']);
      | end
  Lamp224 : Subsystem  DialogController=hmiCreateDDGDialog  mask(MWDashboardBlock){webBlockId=47660420-238c-4dc6-9eb4-f9068d869cf5, webBlockType=lamp, ShowInLibBrowser=on, ShowInitialText=on, HMISrcModelName=[]}
      mask prompts: webBlockType "WebBlock Type"; HMISrcModelName "Source Model"
      mask Help: helpview([docroot '/mapfiles/simulink.map'], 'hmi_lamp')
      mask Display:
      | if strcmp(get_param(bdroot(gcb),'BlockDiagramType'), 'library')
      |     image([(matlabroot) '/toolbox/simulink/hmi/icons/Lamp.png']);
      | end
  Lamp225 : Subsystem  DialogController=hmiCreateDDGDialog  mask(MWDashboardBlock){webBlockId=90219573-4d5f-4979-8dce-527301461ef3, webBlockType=lamp, ShowInLibBrowser=on, ShowInitialText=on, HMISrcModelName=[]}
      mask prompts: webBlockType "WebBlock Type"; HMISrcModelName "Source Model"
      mask Help: helpview([docroot '/mapfiles/simulink.map'], 'hmi_lamp')
      mask Display:
      | if strcmp(get_param(bdroot(gcb),'BlockDiagramType'), 'library')
      |     image([(matlabroot) '/toolbox/simulink/hmi/icons/Lamp.png']);
      | end
  Lamp226 : Subsystem  DialogController=hmiCreateDDGDialog  mask(MWDashboardBlock){webBlockId=a715b041-50eb-478e-b11c-81edf2642573, webBlockType=lamp, ShowInLibBrowser=on, ShowInitialText=on, HMISrcModelName=[]}
      mask prompts: webBlockType "WebBlock Type"; HMISrcModelName "Source Model"
      mask Help: helpview([docroot '/mapfiles/simulink.map'], 'hmi_lamp')
      mask Display:
      | if strcmp(get_param(bdroot(gcb),'BlockDiagramType'), 'library')
      |     image([(matlabroot) '/toolbox/simulink/hmi/icons/Lamp.png']);
      | end
  Lamp227 : Subsystem  DialogController=hmiCreateDDGDialog  mask(MWDashboardBlock){webBlockId=4a6520ff-bedd-4409-a82b-36914affe35f, webBlockType=lamp, ShowInLibBrowser=on, ShowInitialText=on, HMISrcModelName=[]}
      mask prompts: webBlockType "WebBlock Type"; HMISrcModelName "Source Model"
      mask Help: helpview([docroot '/mapfiles/simulink.map'], 'hmi_lamp')
      mask Display:
      | if strcmp(get_param(bdroot(gcb),'BlockDiagramType'), 'library')
      |     image([(matlabroot) '/toolbox/simulink/hmi/icons/Lamp.png']);
      | end
  Lamp228 : Subsystem  DialogController=hmiCreateDDGDialog  mask(MWDashboardBlock){webBlockId=547906fb-3886-4647-bcaf-209b0874f6cf, webBlockType=lamp, ShowInLibBrowser=on, ShowInitialText=on, HMISrcModelName=[]}
      mask prompts: webBlockType "WebBlock Type"; HMISrcModelName "Source Model"
      mask Help: helpview([docroot '/mapfiles/simulink.map'], 'hmi_lamp')
      mask Display:
      | if strcmp(get_param(bdroot(gcb),'BlockDiagramType'), 'library')
      |     image([(matlabroot) '/toolbox/simulink/hmi/icons/Lamp.png']);
      | end
  Lamp229 : Subsystem  DialogController=hmiCreateDDGDialog  mask(MWDashboardBlock){webBlockId=fdb67eec-93d3-4698-acad-5c946660f51b, webBlockType=lamp, ShowInLibBrowser=on, ShowInitialText=on, HMISrcModelName=[]}
      mask prompts: webBlockType "WebBlock Type"; HMISrcModelName "Source Model"
      mask Help: helpview([docroot '/mapfiles/simulink.map'], 'hmi_lamp')
      mask Display:
      | if strcmp(get_param(bdroot(gcb),'BlockDiagramType'), 'library')
      |     image([(matlabroot) '/toolbox/simulink/hmi/icons/Lamp.png']);
      | end
  Lamp23 : Subsystem  DialogController=hmiCreateDDGDialog  mask(MWDashboardBlock){webBlockId=6fd18dd5-ccc1-4345-83e4-14a7d4849f72, webBlockType=lamp, ShowInLibBrowser=on, ShowInitialText=on, HMISrcModelName=[]}
      mask prompts: webBlockType "WebBlock Type"; HMISrcModelName "Source Model"
      mask Help: helpview([docroot '/mapfiles/simulink.map'], 'hmi_lamp')
      mask Display:
      | if strcmp(get_param(bdroot(gcb),'BlockDiagramType'), 'library')
      |     image([(matlabroot) '/toolbox/simulink/hmi/icons/Lamp.png']);
      | end
  Lamp230 : Subsystem  DialogController=hmiCreateDDGDialog  mask(MWDashboardBlock){webBlockId=fab56aa1-f8be-4329-acc7-1c42950c617d, webBlockType=lamp, ShowInLibBrowser=on, ShowInitialText=on, HMISrcModelName=[]}
      mask prompts: webBlockType "WebBlock Type"; HMISrcModelName "Source Model"
      mask Help: helpview([docroot '/mapfiles/simulink.map'], 'hmi_lamp')
      mask Display:
      | if strcmp(get_param(bdroot(gcb),'BlockDiagramType'), 'library')
      |     image([(matlabroot) '/toolbox/simulink/hmi/icons/Lamp.png']);
      | end
  Lamp231 : Subsystem  DialogController=hmiCreateDDGDialog  mask(MWDashboardBlock){webBlockId=35212785-7817-4db9-88a7-c5ffbe5d9cab, webBlockType=lamp, ShowInLibBrowser=on, ShowInitialText=on, HMISrcModelName=[]}
      mask prompts: webBlockType "WebBlock Type"; HMISrcModelName "Source Model"
      mask Help: helpview([docroot '/mapfiles/simulink.map'], 'hmi_lamp')
      mask Display:
      | if strcmp(get_param(bdroot(gcb),'BlockDiagramType'), 'library')
      |     image([(matlabroot) '/toolbox/simulink/hmi/icons/Lamp.png']);
      | end
  Lamp232 : Subsystem  DialogController=hmiCreateDDGDialog  mask(MWDashboardBlock){webBlockId=36db3cb5-26d2-472e-aec2-112568d8e6eb, webBlockType=lamp, ShowInLibBrowser=on, ShowInitialText=on, HMISrcModelName=[]}
      mask prompts: webBlockType "WebBlock Type"; HMISrcModelName "Source Model"
      mask Help: helpview([docroot '/mapfiles/simulink.map'], 'hmi_lamp')
      mask Display:
      | if strcmp(get_param(bdroot(gcb),'BlockDiagramType'), 'library')
      |     image([(matlabroot) '/toolbox/simulink/hmi/icons/Lamp.png']);
      | end
  Lamp233 : Subsystem  DialogController=hmiCreateDDGDialog  mask(MWDashboardBlock){webBlockId=23a8a3ea-62df-42a8-b044-deb824019a68, webBlockType=lamp, ShowInLibBrowser=on, ShowInitialText=on, HMISrcModelName=[]}
      mask prompts: webBlockType "WebBlock Type"; HMISrcModelName "Source Model"
      mask Help: helpview([docroot '/mapfiles/simulink.map'], 'hmi_lamp')
      mask Display:
      | if strcmp(get_param(bdroot(gcb),'BlockDiagramType'), 'library')
      |     image([(matlabroot) '/toolbox/simulink/hmi/icons/Lamp.png']);
      | end
  Lamp234 : Subsystem  DialogController=hmiCreateDDGDialog  mask(MWDashboardBlock){webBlockId=6ed5e14d-673b-45c9-8b50-e1f64a2c1b1a, webBlockType=lamp, ShowInLibBrowser=on, ShowInitialText=on, HMISrcModelName=[]}
      mask prompts: webBlockType "WebBlock Type"; HMISrcModelName "Source Model"
      mask Help: helpview([docroot '/mapfiles/simulink.map'], 'hmi_lamp')
      mask Display:
      | if strcmp(get_param(bdroot(gcb),'BlockDiagramType'), 'library')
      |     image([(matlabroot) '/toolbox/simulink/hmi/icons/Lamp.png']);
      | end
  Lamp235 : Subsystem  DialogController=hmiCreateDDGDialog  mask(MWDashboardBlock){webBlockId=ccd3903d-227f-42db-b4e0-646030c36695, webBlockType=lamp, ShowInLibBrowser=on, ShowInitialText=on, HMISrcModelName=[]}
      mask prompts: webBlockType "WebBlock Type"; HMISrcModelName "Source Model"
      mask Help: helpview([docroot '/mapfiles/simulink.map'], 'hmi_lamp')
      mask Display:
      | if strcmp(get_param(bdroot(gcb),'BlockDiagramType'), 'library')
      |     image([(matlabroot) '/toolbox/simulink/hmi/icons/Lamp.png']);
      | end
  Lamp236 : Subsystem  DialogController=hmiCreateDDGDialog  mask(MWDashboardBlock){webBlockId=11d42446-51f7-485f-9a9e-cfafa2593298, webBlockType=lamp, ShowInLibBrowser=on, ShowInitialText=on, HMISrcModelName=[]}
      mask prompts: webBlockType "WebBlock Type"; HMISrcModelName "Source Model"
      mask Help: helpview([docroot '/mapfiles/simulink.map'], 'hmi_lamp')
      mask Display:
      | if strcmp(get_param(bdroot(gcb),'BlockDiagramType'), 'library')
      |     image([(matlabroot) '/toolbox/simulink/hmi/icons/Lamp.png']);
      | end
  Lamp237 : Subsystem  DialogController=hmiCreateDDGDialog  mask(MWDashboardBlock){webBlockId=b54e4086-7937-4f1e-999e-b8a33efa6ad3, webBlockType=lamp, ShowInLibBrowser=on, ShowInitialText=on, HMISrcModelName=[]}
      mask prompts: webBlockType "WebBlock Type"; HMISrcModelName "Source Model"
      mask Help: helpview([docroot '/mapfiles/simulink.map'], 'hmi_lamp')
      mask Display:
      | if strcmp(get_param(bdroot(gcb),'BlockDiagramType'), 'library')
      |     image([(matlabroot) '/toolbox/simulink/hmi/icons/Lamp.png']);
      | end
  Lamp238 : Subsystem  DialogController=hmiCreateDDGDialog  mask(MWDashboardBlock){webBlockId=127b46dd-9deb-4e5d-a286-ec1f496b8cf9, webBlockType=lamp, ShowInLibBrowser=on, ShowInitialText=on, HMISrcModelName=[]}
      mask prompts: webBlockType "WebBlock Type"; HMISrcModelName "Source Model"
      mask Help: helpview([docroot '/mapfiles/simulink.map'], 'hmi_lamp')
      mask Display:
      | if strcmp(get_param(bdroot(gcb),'BlockDiagramType'), 'library')
      |     image([(matlabroot) '/toolbox/simulink/hmi/icons/Lamp.png']);
      | end
  Lamp239 : Subsystem  DialogController=hmiCreateDDGDialog  mask(MWDashboardBlock){webBlockId=cffaf9c3-ccf6-434a-a642-d214c57e9279, webBlockType=lamp, ShowInLibBrowser=on, ShowInitialText=on, HMISrcModelName=[]}
      mask prompts: webBlockType "WebBlock Type"; HMISrcModelName "Source Model"
      mask Help: helpview([docroot '/mapfiles/simulink.map'], 'hmi_lamp')
      mask Display:
      | if strcmp(get_param(bdroot(gcb),'BlockDiagramType'), 'library')
      |     image([(matlabroot) '/toolbox/simulink/hmi/icons/Lamp.png']);
      | end
  Lamp24 : Subsystem  DialogController=hmiCreateDDGDialog  mask(MWDashboardBlock){webBlockId=4ab3ce86-100a-4ddf-b5c0-c02a365c70e4, webBlockType=lamp, ShowInLibBrowser=on, ShowInitialText=on, HMISrcModelName=[]}
      mask prompts: webBlockType "WebBlock Type"; HMISrcModelName "Source Model"
      mask Help: helpview([docroot '/mapfiles/simulink.map'], 'hmi_lamp')
      mask Display:
      | if strcmp(get_param(bdroot(gcb),'BlockDiagramType'), 'library')
      |     image([(matlabroot) '/toolbox/simulink/hmi/icons/Lamp.png']);
      | end
  Lamp240 : Subsystem  DialogController=hmiCreateDDGDialog  mask(MWDashboardBlock){webBlockId=3d8ef522-7a13-4a57-bef3-3eca10ba0861, webBlockType=lamp, ShowInLibBrowser=on, ShowInitialText=on, HMISrcModelName=[]}
      mask prompts: webBlockType "WebBlock Type"; HMISrcModelName "Source Model"
      mask Help: helpview([docroot '/mapfiles/simulink.map'], 'hmi_lamp')
      mask Display:
      | if strcmp(get_param(bdroot(gcb),'BlockDiagramType'), 'library')
      |     image([(matlabroot) '/toolbox/simulink/hmi/icons/Lamp.png']);
      | end
  Lamp241 : Subsystem  DialogController=hmiCreateDDGDialog  mask(MWDashboardBlock){webBlockId=38071224-ca3b-4c31-a6d3-da565f7248b9, webBlockType=lamp, ShowInLibBrowser=on, ShowInitialText=on, HMISrcModelName=[]}
      mask prompts: webBlockType "WebBlock Type"; HMISrcModelName "Source Model"
      mask Help: helpview([docroot '/mapfiles/simulink.map'], 'hmi_lamp')
      mask Display:
      | if strcmp(get_param(bdroot(gcb),'BlockDiagramType'), 'library')
      |     image([(matlabroot) '/toolbox/simulink/hmi/icons/Lamp.png']);
      | end
  Lamp242 : Subsystem  DialogController=hmiCreateDDGDialog  mask(MWDashboardBlock){webBlockId=58ff1269-242b-4fc7-851d-58061b07164f, webBlockType=lamp, ShowInLibBrowser=on, ShowInitialText=on, HMISrcModelName=[]}
      mask prompts: webBlockType "WebBlock Type"; HMISrcModelName "Source Model"
      mask Help: helpview([docroot '/mapfiles/simulink.map'], 'hmi_lamp')
      mask Display:
      | if strcmp(get_param(bdroot(gcb),'BlockDiagramType'), 'library')
      |     image([(matlabroot) '/toolbox/simulink/hmi/icons/Lamp.png']);
      | end
  Lamp243 : Subsystem  DialogController=hmiCreateDDGDialog  mask(MWDashboardBlock){webBlockId=66d463ee-c297-4024-b06b-96f62c7cb880, webBlockType=lamp, ShowInLibBrowser=on, ShowInitialText=on, HMISrcModelName=[]}
      mask prompts: webBlockType "WebBlock Type"; HMISrcModelName "Source Model"
      mask Help: helpview([docroot '/mapfiles/simulink.map'], 'hmi_lamp')
      mask Display:
      | if strcmp(get_param(bdroot(gcb),'BlockDiagramType'), 'library')
      |     image([(matlabroot) '/toolbox/simulink/hmi/icons/Lamp.png']);
      | end
  Lamp244 : Subsystem  DialogController=hmiCreateDDGDialog  mask(MWDashboardBlock){webBlockId=c28dea58-9212-499c-9bcd-0d4c794592a5, webBlockType=lamp, ShowInLibBrowser=on, ShowInitialText=on, HMISrcModelName=[]}
      mask prompts: webBlockType "WebBlock Type"; HMISrcModelName "Source Model"
      mask Help: helpview([docroot '/mapfiles/simulink.map'], 'hmi_lamp')
      mask Display:
      | if strcmp(get_param(bdroot(gcb),'BlockDiagramType'), 'library')
      |     image([(matlabroot) '/toolbox/simulink/hmi/icons/Lamp.png']);
      | end
  Lamp245 : Subsystem  DialogController=hmiCreateDDGDialog  mask(MWDashboardBlock){webBlockId=d8cfae6a-a053-47b0-aa20-6cc2be88b82a, webBlockType=lamp, ShowInLibBrowser=on, ShowInitialText=on, HMISrcModelName=[]}
      mask prompts: webBlockType "WebBlock Type"; HMISrcModelName "Source Model"
      mask Help: helpview([docroot '/mapfiles/simulink.map'], 'hmi_lamp')
      mask Display:
      | if strcmp(get_param(bdroot(gcb),'BlockDiagramType'), 'library')
      |     image([(matlabroot) '/toolbox/simulink/hmi/icons/Lamp.png']);
      | end
  Lamp246 : Subsystem  DialogController=hmiCreateDDGDialog  mask(MWDashboardBlock){webBlockId=fdf7b163-5b7d-4948-bc42-9e1565ff7527, webBlockType=lamp, ShowInLibBrowser=on, ShowInitialText=on, HMISrcModelName=[]}
      mask prompts: webBlockType "WebBlock Type"; HMISrcModelName "Source Model"
      mask Help: helpview([docroot '/mapfiles/simulink.map'], 'hmi_lamp')
      mask Display:
      | if strcmp(get_param(bdroot(gcb),'BlockDiagramType'), 'library')
      |     image([(matlabroot) '/toolbox/simulink/hmi/icons/Lamp.png']);
      | end
  Lamp247 : Subsystem  DialogController=hmiCreateDDGDialog  mask(MWDashboardBlock){webBlockId=6ffacc3e-5747-40ad-86a3-971bd636c5e9, webBlockType=lamp, ShowInLibBrowser=on, ShowInitialText=on, HMISrcModelName=[]}
      mask prompts: webBlockType "WebBlock Type"; HMISrcModelName "Source Model"
      mask Help: helpview([docroot '/mapfiles/simulink.map'], 'hmi_lamp')
      mask Display:
      | if strcmp(get_param(bdroot(gcb),'BlockDiagramType'), 'library')
      |     image([(matlabroot) '/toolbox/simulink/hmi/icons/Lamp.png']);
      | end
  Lamp248 : Subsystem  DialogController=hmiCreateDDGDialog  mask(MWDashboardBlock){webBlockId=d9c1cdab-d408-45c9-981f-7cd4b3946912, webBlockType=lamp, ShowInLibBrowser=on, ShowInitialText=on, HMISrcModelName=[]}
      mask prompts: webBlockType "WebBlock Type"; HMISrcModelName "Source Model"
      mask Help: helpview([docroot '/mapfiles/simulink.map'], 'hmi_lamp')
      mask Display:
      | if strcmp(get_param(bdroot(gcb),'BlockDiagramType'), 'library')
      |     image([(matlabroot) '/toolbox/simulink/hmi/icons/Lamp.png']);
      | end
  Lamp249 : Subsystem  DialogController=hmiCreateDDGDialog  mask(MWDashboardBlock){webBlockId=00d9a3e0-9c04-429d-9aea-69c6a2a7046b, webBlockType=lamp, ShowInLibBrowser=on, ShowInitialText=on, HMISrcModelName=[]}
      mask prompts: webBlockType "WebBlock Type"; HMISrcModelName "Source Model"
      mask Help: helpview([docroot '/mapfiles/simulink.map'], 'hmi_lamp')
      mask Display:
      | if strcmp(get_param(bdroot(gcb),'BlockDiagramType'), 'library')
      |     image([(matlabroot) '/toolbox/simulink/hmi/icons/Lamp.png']);
      | end
  Lamp25 : Subsystem  DialogController=hmiCreateDDGDialog  mask(MWDashboardBlock){webBlockId=f0c2663f-36da-4fa1-aa17-4f11596c3e71, webBlockType=lamp, ShowInLibBrowser=on, ShowInitialText=on, HMISrcModelName=[]}
      mask prompts: webBlockType "WebBlock Type"; HMISrcModelName "Source Model"
      mask Help: helpview([docroot '/mapfiles/simulink.map'], 'hmi_lamp')
      mask Display:
      | if strcmp(get_param(bdroot(gcb),'BlockDiagramType'), 'library')
      |     image([(matlabroot) '/toolbox/simulink/hmi/icons/Lamp.png']);
      | end
  Lamp250 : Subsystem  DialogController=hmiCreateDDGDialog  mask(MWDashboardBlock){webBlockId=01818d76-86c3-464a-a5ab-c236fc3deda3, webBlockType=lamp, ShowInLibBrowser=on, ShowInitialText=on, HMISrcModelName=[]}
      mask prompts: webBlockType "WebBlock Type"; HMISrcModelName "Source Model"
      mask Help: helpview([docroot '/mapfiles/simulink.map'], 'hmi_lamp')
      mask Display:
      | if strcmp(get_param(bdroot(gcb),'BlockDiagramType'), 'library')
      |     image([(matlabroot) '/toolbox/simulink/hmi/icons/Lamp.png']);
      | end
  Lamp251 : Subsystem  DialogController=hmiCreateDDGDialog  mask(MWDashboardBlock){webBlockId=d56bd736-c2a0-4a77-8ef3-e4d9f1a8f836, webBlockType=lamp, ShowInLibBrowser=on, ShowInitialText=on, HMISrcModelName=[]}
      mask prompts: webBlockType "WebBlock Type"; HMISrcModelName "Source Model"
      mask Help: helpview([docroot '/mapfiles/simulink.map'], 'hmi_lamp')
      mask Display:
      | if strcmp(get_param(bdroot(gcb),'BlockDiagramType'), 'library')
      |     image([(matlabroot) '/toolbox/simulink/hmi/icons/Lamp.png']);
      | end
  Lamp252 : Subsystem  DialogController=hmiCreateDDGDialog  mask(MWDashboardBlock){webBlockId=35caff30-d7ed-4681-ad87-2fd31df76396, webBlockType=lamp, ShowInLibBrowser=on, ShowInitialText=on, HMISrcModelName=[]}
      mask prompts: webBlockType "WebBlock Type"; HMISrcModelName "Source Model"
      mask Help: helpview([docroot '/mapfiles/simulink.map'], 'hmi_lamp')
      mask Display:
      | if strcmp(get_param(bdroot(gcb),'BlockDiagramType'), 'library')
      |     image([(matlabroot) '/toolbox/simulink/hmi/icons/Lamp.png']);
      | end
  Lamp253 : Subsystem  DialogController=hmiCreateDDGDialog  mask(MWDashboardBlock){webBlockId=02f98fb0-0e93-48a2-aab1-0e5fd4546772, webBlockType=lamp, ShowInLibBrowser=on, ShowInitialText=on, HMISrcModelName=[]}
      mask prompts: webBlockType "WebBlock Type"; HMISrcModelName "Source Model"
      mask Help: helpview([docroot '/mapfiles/simulink.map'], 'hmi_lamp')
      mask Display:
      | if strcmp(get_param(bdroot(gcb),'BlockDiagramType'), 'library')
      |     image([(matlabroot) '/toolbox/simulink/hmi/icons/Lamp.png']);
      | end
  Lamp254 : Subsystem  DialogController=hmiCreateDDGDialog  mask(MWDashboardBlock){webBlockId=4e36052a-95be-4474-a601-7562eaf60572, webBlockType=lamp, ShowInLibBrowser=on, ShowInitialText=on, HMISrcModelName=[]}
      mask prompts: webBlockType "WebBlock Type"; HMISrcModelName "Source Model"
      mask Help: helpview([docroot '/mapfiles/simulink.map'], 'hmi_lamp')
      mask Display:
      | if strcmp(get_param(bdroot(gcb),'BlockDiagramType'), 'library')
      |     image([(matlabroot) '/toolbox/simulink/hmi/icons/Lamp.png']);
      | end
  Lamp255 : Subsystem  DialogController=hmiCreateDDGDialog  mask(MWDashboardBlock){webBlockId=229cde54-e6ae-4346-9341-45dedd22f826, webBlockType=lamp, ShowInLibBrowser=on, ShowInitialText=on, HMISrcModelName=[]}
      mask prompts: webBlockType "WebBlock Type"; HMISrcModelName "Source Model"
      mask Help: helpview([docroot '/mapfiles/simulink.map'], 'hmi_lamp')
      mask Display:
      | if strcmp(get_param(bdroot(gcb),'BlockDiagramType'), 'library')
      |     image([(matlabroot) '/toolbox/simulink/hmi/icons/Lamp.png']);
      | end
  Lamp26 : Subsystem  DialogController=hmiCreateDDGDialog  mask(MWDashboardBlock){webBlockId=f3a87a4f-3c7c-4ce8-950d-375e97aafbf2, webBlockType=lamp, ShowInLibBrowser=on, ShowInitialText=on, HMISrcModelName=[]}
      mask prompts: webBlockType "WebBlock Type"; HMISrcModelName "Source Model"
      mask Help: helpview([docroot '/mapfiles/simulink.map'], 'hmi_lamp')
      mask Display:
      | if strcmp(get_param(bdroot(gcb),'BlockDiagramType'), 'library')
      |     image([(matlabroot) '/toolbox/simulink/hmi/icons/Lamp.png']);
      | end
  Lamp27 : Subsystem  DialogController=hmiCreateDDGDialog  mask(MWDashboardBlock){webBlockId=6f288dfc-0d46-4007-b9f6-68ee6e3bc138, webBlockType=lamp, ShowInLibBrowser=on, ShowInitialText=on, HMISrcModelName=[]}
      mask prompts: webBlockType "WebBlock Type"; HMISrcModelName "Source Model"
      mask Help: helpview([docroot '/mapfiles/simulink.map'], 'hmi_lamp')
      mask Display:
      | if strcmp(get_param(bdroot(gcb),'BlockDiagramType'), 'library')
      |     image([(matlabroot) '/toolbox/simulink/hmi/icons/Lamp.png']);
      | end
  Lamp28 : Subsystem  DialogController=hmiCreateDDGDialog  mask(MWDashboardBlock){webBlockId=0733f91a-c916-4329-b38b-30b8efaf5ec0, webBlockType=lamp, ShowInLibBrowser=on, ShowInitialText=on, HMISrcModelName=[]}
      mask prompts: webBlockType "WebBlock Type"; HMISrcModelName "Source Model"
      mask Help: helpview([docroot '/mapfiles/simulink.map'], 'hmi_lamp')
      mask Display:
      | if strcmp(get_param(bdroot(gcb),'BlockDiagramType'), 'library')
      |     image([(matlabroot) '/toolbox/simulink/hmi/icons/Lamp.png']);
      | end
  Lamp29 : Subsystem  DialogController=hmiCreateDDGDialog  mask(MWDashboardBlock){webBlockId=df8aeb41-aa18-4bbf-b946-328db1edaad5, webBlockType=lamp, ShowInLibBrowser=on, ShowInitialText=on, HMISrcModelName=[]}
      mask prompts: webBlockType "WebBlock Type"; HMISrcModelName "Source Model"
      mask Help: helpview([docroot '/mapfiles/simulink.map'], 'hmi_lamp')
      mask Display:
      | if strcmp(get_param(bdroot(gcb),'BlockDiagramType'), 'library')
      |     image([(matlabroot) '/toolbox/simulink/hmi/icons/Lamp.png']);
      | end
  Lamp3 : Subsystem  DialogController=hmiCreateDDGDialog  mask(MWDashboardBlock){webBlockId=d138b7a7-16bf-4dc3-b99c-c782157d3ab8, webBlockType=lamp, ShowInLibBrowser=on, ShowInitialText=on, HMISrcModelName=[]}
      mask prompts: webBlockType "WebBlock Type"; HMISrcModelName "Source Model"
      mask Help: helpview([docroot '/mapfiles/simulink.map'], 'hmi_lamp')
      mask Display:
      | if strcmp(get_param(bdroot(gcb),'BlockDiagramType'), 'library')
      |     image([(matlabroot) '/toolbox/simulink/hmi/icons/Lamp.png']);
      | end
  Lamp30 : Subsystem  DialogController=hmiCreateDDGDialog  mask(MWDashboardBlock){webBlockId=4b0fd869-d52a-48d4-ac27-3c42dd56d697, webBlockType=lamp, ShowInLibBrowser=on, ShowInitialText=on, HMISrcModelName=[]}
      mask prompts: webBlockType "WebBlock Type"; HMISrcModelName "Source Model"
      mask Help: helpview([docroot '/mapfiles/simulink.map'], 'hmi_lamp')
      mask Display:
      | if strcmp(get_param(bdroot(gcb),'BlockDiagramType'), 'library')
      |     image([(matlabroot) '/toolbox/simulink/hmi/icons/Lamp.png']);
      | end
  Lamp31 : Subsystem  DialogController=hmiCreateDDGDialog  mask(MWDashboardBlock){webBlockId=f9a6e0e5-5df2-47e3-9740-eb00dd27c4a3, webBlockType=lamp, ShowInLibBrowser=on, ShowInitialText=on, HMISrcModelName=[]}
      mask prompts: webBlockType "WebBlock Type"; HMISrcModelName "Source Model"
      mask Help: helpview([docroot '/mapfiles/simulink.map'], 'hmi_lamp')
      mask Display:
      | if strcmp(get_param(bdroot(gcb),'BlockDiagramType'), 'library')
      |     image([(matlabroot) '/toolbox/simulink/hmi/icons/Lamp.png']);
      | end
  Lamp32 : Subsystem  DialogController=hmiCreateDDGDialog  mask(MWDashboardBlock){webBlockId=8ade0b88-ee94-429b-9c30-e7fba9b50aaa, webBlockType=lamp, ShowInLibBrowser=on, ShowInitialText=on, HMISrcModelName=[]}
      mask prompts: webBlockType "WebBlock Type"; HMISrcModelName "Source Model"
      mask Help: helpview([docroot '/mapfiles/simulink.map'], 'hmi_lamp')
      mask Display:
      | if strcmp(get_param(bdroot(gcb),'BlockDiagramType'), 'library')
      |     image([(matlabroot) '/toolbox/simulink/hmi/icons/Lamp.png']);
      | end
  Lamp33 : Subsystem  DialogController=hmiCreateDDGDialog  mask(MWDashboardBlock){webBlockId=a00ce4dd-9f96-4e89-94b5-34a70770e268, webBlockType=lamp, ShowInLibBrowser=on, ShowInitialText=on, HMISrcModelName=[]}
      mask prompts: webBlockType "WebBlock Type"; HMISrcModelName "Source Model"
      mask Help: helpview([docroot '/mapfiles/simulink.map'], 'hmi_lamp')
      mask Display:
      | if strcmp(get_param(bdroot(gcb),'BlockDiagramType'), 'library')
      |     image([(matlabroot) '/toolbox/simulink/hmi/icons/Lamp.png']);
      | end
  Lamp34 : Subsystem  DialogController=hmiCreateDDGDialog  mask(MWDashboardBlock){webBlockId=bff7db60-d371-4bfa-b1f4-c393570249a9, webBlockType=lamp, ShowInLibBrowser=on, ShowInitialText=on, HMISrcModelName=[]}
      mask prompts: webBlockType "WebBlock Type"; HMISrcModelName "Source Model"
      mask Help: helpview([docroot '/mapfiles/simulink.map'], 'hmi_lamp')
      mask Display:
      | if strcmp(get_param(bdroot(gcb),'BlockDiagramType'), 'library')
      |     image([(matlabroot) '/toolbox/simulink/hmi/icons/Lamp.png']);
      | end
  Lamp35 : Subsystem  DialogController=hmiCreateDDGDialog  mask(MWDashboardBlock){webBlockId=956579a1-6fd9-4f6b-8c59-3a2ecc97342d, webBlockType=lamp, ShowInLibBrowser=on, ShowInitialText=on, HMISrcModelName=[]}
      mask prompts: webBlockType "WebBlock Type"; HMISrcModelName "Source Model"
      mask Help: helpview([docroot '/mapfiles/simulink.map'], 'hmi_lamp')
      mask Display:
      | if strcmp(get_param(bdroot(gcb),'BlockDiagramType'), 'library')
      |     image([(matlabroot) '/toolbox/simulink/hmi/icons/Lamp.png']);
      | end
  Lamp36 : Subsystem  DialogController=hmiCreateDDGDialog  mask(MWDashboardBlock){webBlockId=26c375f2-0adc-485a-9a94-cf01a6946415, webBlockType=lamp, ShowInLibBrowser=on, ShowInitialText=on, HMISrcModelName=[]}
      mask prompts: webBlockType "WebBlock Type"; HMISrcModelName "Source Model"
      mask Help: helpview([docroot '/mapfiles/simulink.map'], 'hmi_lamp')
      mask Display:
      | if strcmp(get_param(bdroot(gcb),'BlockDiagramType'), 'library')
      |     image([(matlabroot) '/toolbox/simulink/hmi/icons/Lamp.png']);
      | end
  Lamp37 : Subsystem  DialogController=hmiCreateDDGDialog  mask(MWDashboardBlock){webBlockId=64d85fa5-2154-45dd-b6b3-8edcab9cf7f8, webBlockType=lamp, ShowInLibBrowser=on, ShowInitialText=on, HMISrcModelName=[]}
      mask prompts: webBlockType "WebBlock Type"; HMISrcModelName "Source Model"
      mask Help: helpview([docroot '/mapfiles/simulink.map'], 'hmi_lamp')
      mask Display:
      | if strcmp(get_param(bdroot(gcb),'BlockDiagramType'), 'library')
      |     image([(matlabroot) '/toolbox/simulink/hmi/icons/Lamp.png']);
      | end
  Lamp38 : Subsystem  DialogController=hmiCreateDDGDialog  mask(MWDashboardBlock){webBlockId=76646e42-c804-4623-b5ae-7115381d90c4, webBlockType=lamp, ShowInLibBrowser=on, ShowInitialText=on, HMISrcModelName=[]}
      mask prompts: webBlockType "WebBlock Type"; HMISrcModelName "Source Model"
      mask Help: helpview([docroot '/mapfiles/simulink.map'], 'hmi_lamp')
      mask Display:
      | if strcmp(get_param(bdroot(gcb),'BlockDiagramType'), 'library')
      |     image([(matlabroot) '/toolbox/simulink/hmi/icons/Lamp.png']);
      | end
  Lamp39 : Subsystem  DialogController=hmiCreateDDGDialog  mask(MWDashboardBlock){webBlockId=00d5d4f2-f6d4-405b-a6db-3bbba86988b7, webBlockType=lamp, ShowInLibBrowser=on, ShowInitialText=on, HMISrcModelName=[]}
      mask prompts: webBlockType "WebBlock Type"; HMISrcModelName "Source Model"
      mask Help: helpview([docroot '/mapfiles/simulink.map'], 'hmi_lamp')
      mask Display:
      | if strcmp(get_param(bdroot(gcb),'BlockDiagramType'), 'library')
      |     image([(matlabroot) '/toolbox/simulink/hmi/icons/Lamp.png']);
      | end
  Lamp4 : Subsystem  DialogController=hmiCreateDDGDialog  mask(MWDashboardBlock){webBlockId=026a4e90-ca77-41c1-9927-6f4cf3af978c, webBlockType=lamp, ShowInLibBrowser=on, ShowInitialText=on, HMISrcModelName=[]}
      mask prompts: webBlockType "WebBlock Type"; HMISrcModelName "Source Model"
      mask Help: helpview([docroot '/mapfiles/simulink.map'], 'hmi_lamp')
      mask Display:
      | if strcmp(get_param(bdroot(gcb),'BlockDiagramType'), 'library')
      |     image([(matlabroot) '/toolbox/simulink/hmi/icons/Lamp.png']);
      | end
  Lamp40 : Subsystem  DialogController=hmiCreateDDGDialog  mask(MWDashboardBlock){webBlockId=628cc884-58bc-4f20-88d4-a394f5fb1bd7, webBlockType=lamp, ShowInLibBrowser=on, ShowInitialText=on, HMISrcModelName=[]}
      mask prompts: webBlockType "WebBlock Type"; HMISrcModelName "Source Model"
      mask Help: helpview([docroot '/mapfiles/simulink.map'], 'hmi_lamp')
      mask Display:
      | if strcmp(get_param(bdroot(gcb),'BlockDiagramType'), 'library')
      |     image([(matlabroot) '/toolbox/simulink/hmi/icons/Lamp.png']);
      | end
  Lamp41 : Subsystem  DialogController=hmiCreateDDGDialog  mask(MWDashboardBlock){webBlockId=8a851000-20b5-4dc6-9a58-a1f85ae57a4a, webBlockType=lamp, ShowInLibBrowser=on, ShowInitialText=on, HMISrcModelName=[]}
      mask prompts: webBlockType "WebBlock Type"; HMISrcModelName "Source Model"
      mask Help: helpview([docroot '/mapfiles/simulink.map'], 'hmi_lamp')
      mask Display:
      | if strcmp(get_param(bdroot(gcb),'BlockDiagramType'), 'library')
      |     image([(matlabroot) '/toolbox/simulink/hmi/icons/Lamp.png']);
      | end
  Lamp42 : Subsystem  DialogController=hmiCreateDDGDialog  mask(MWDashboardBlock){webBlockId=3c8a8182-d810-45a3-9371-cf566097a3bd, webBlockType=lamp, ShowInLibBrowser=on, ShowInitialText=on, HMISrcModelName=[]}
      mask prompts: webBlockType "WebBlock Type"; HMISrcModelName "Source Model"
      mask Help: helpview([docroot '/mapfiles/simulink.map'], 'hmi_lamp')
      mask Display:
      | if strcmp(get_param(bdroot(gcb),'BlockDiagramType'), 'library')
      |     image([(matlabroot) '/toolbox/simulink/hmi/icons/Lamp.png']);
      | end
  Lamp43 : Subsystem  DialogController=hmiCreateDDGDialog  mask(MWDashboardBlock){webBlockId=46c1efe7-f13f-49fc-b7f2-bd1c61c35c8e, webBlockType=lamp, ShowInLibBrowser=on, ShowInitialText=on, HMISrcModelName=[]}
      mask prompts: webBlockType "WebBlock Type"; HMISrcModelName "Source Model"
      mask Help: helpview([docroot '/mapfiles/simulink.map'], 'hmi_lamp')
      mask Display:
      | if strcmp(get_param(bdroot(gcb),'BlockDiagramType'), 'library')
      |     image([(matlabroot) '/toolbox/simulink/hmi/icons/Lamp.png']);
      | end
  Lamp44 : Subsystem  DialogController=hmiCreateDDGDialog  mask(MWDashboardBlock){webBlockId=674aed14-18bd-49d3-825e-b9fff561bcda, webBlockType=lamp, ShowInLibBrowser=on, ShowInitialText=on, HMISrcModelName=[]}
      mask prompts: webBlockType "WebBlock Type"; HMISrcModelName "Source Model"
      mask Help: helpview([docroot '/mapfiles/simulink.map'], 'hmi_lamp')
      mask Display:
      | if strcmp(get_param(bdroot(gcb),'BlockDiagramType'), 'library')
      |     image([(matlabroot) '/toolbox/simulink/hmi/icons/Lamp.png']);
      | end
  Lamp45 : Subsystem  DialogController=hmiCreateDDGDialog  mask(MWDashboardBlock){webBlockId=8434b90b-e9da-4ee0-baac-8e48445e33dc, webBlockType=lamp, ShowInLibBrowser=on, ShowInitialText=on, HMISrcModelName=[]}
      mask prompts: webBlockType "WebBlock Type"; HMISrcModelName "Source Model"
      mask Help: helpview([docroot '/mapfiles/simulink.map'], 'hmi_lamp')
      mask Display:
      | if strcmp(get_param(bdroot(gcb),'BlockDiagramType'), 'library')
      |     image([(matlabroot) '/toolbox/simulink/hmi/icons/Lamp.png']);
      | end
  Lamp46 : Subsystem  DialogController=hmiCreateDDGDialog  mask(MWDashboardBlock){webBlockId=fe968753-1ef9-4d59-b96a-ea9fdb486e8b, webBlockType=lamp, ShowInLibBrowser=on, ShowInitialText=on, HMISrcModelName=[]}
      mask prompts: webBlockType "WebBlock Type"; HMISrcModelName "Source Model"
      mask Help: helpview([docroot '/mapfiles/simulink.map'], 'hmi_lamp')
      mask Display:
      | if strcmp(get_param(bdroot(gcb),'BlockDiagramType'), 'library')
      |     image([(matlabroot) '/toolbox/simulink/hmi/icons/Lamp.png']);
      | end
  Lamp47 : Subsystem  DialogController=hmiCreateDDGDialog  mask(MWDashboardBlock){webBlockId=8d7913d0-b3ef-4816-b568-beeb172bf3c8, webBlockType=lamp, ShowInLibBrowser=on, ShowInitialText=on, HMISrcModelName=[]}
      mask prompts: webBlockType "WebBlock Type"; HMISrcModelName "Source Model"
      mask Help: helpview([docroot '/mapfiles/simulink.map'], 'hmi_lamp')
      mask Display:
      | if strcmp(get_param(bdroot(gcb),'BlockDiagramType'), 'library')
      |     image([(matlabroot) '/toolbox/simulink/hmi/icons/Lamp.png']);
      | end
  Lamp48 : Subsystem  DialogController=hmiCreateDDGDialog  mask(MWDashboardBlock){webBlockId=704c1d0a-d2d2-41dd-97c8-1119502ff3b8, webBlockType=lamp, ShowInLibBrowser=on, ShowInitialText=on, HMISrcModelName=[]}
      mask prompts: webBlockType "WebBlock Type"; HMISrcModelName "Source Model"
      mask Help: helpview([docroot '/mapfiles/simulink.map'], 'hmi_lamp')
      mask Display:
      | if strcmp(get_param(bdroot(gcb),'BlockDiagramType'), 'library')
      |     image([(matlabroot) '/toolbox/simulink/hmi/icons/Lamp.png']);
      | end
  Lamp49 : Subsystem  DialogController=hmiCreateDDGDialog  mask(MWDashboardBlock){webBlockId=624cc51e-8b57-41bf-847b-262d22a1d9a2, webBlockType=lamp, ShowInLibBrowser=on, ShowInitialText=on, HMISrcModelName=[]}
      mask prompts: webBlockType "WebBlock Type"; HMISrcModelName "Source Model"
      mask Help: helpview([docroot '/mapfiles/simulink.map'], 'hmi_lamp')
      mask Display:
      | if strcmp(get_param(bdroot(gcb),'BlockDiagramType'), 'library')
      |     image([(matlabroot) '/toolbox/simulink/hmi/icons/Lamp.png']);
      | end
  Lamp5 : Subsystem  DialogController=hmiCreateDDGDialog  mask(MWDashboardBlock){webBlockId=dc366348-e489-4435-aa09-ee8f2036b1a6, webBlockType=lamp, ShowInLibBrowser=on, ShowInitialText=on, HMISrcModelName=[]}
      mask prompts: webBlockType "WebBlock Type"; HMISrcModelName "Source Model"
      mask Help: helpview([docroot '/mapfiles/simulink.map'], 'hmi_lamp')
      mask Display:
      | if strcmp(get_param(bdroot(gcb),'BlockDiagramType'), 'library')
      |     image([(matlabroot) '/toolbox/simulink/hmi/icons/Lamp.png']);
      | end
  Lamp50 : Subsystem  DialogController=hmiCreateDDGDialog  mask(MWDashboardBlock){webBlockId=7126e2d8-4fb7-46d7-ac84-74269e524865, webBlockType=lamp, ShowInLibBrowser=on, ShowInitialText=on, HMISrcModelName=[]}
      mask prompts: webBlockType "WebBlock Type"; HMISrcModelName "Source Model"
      mask Help: helpview([docroot '/mapfiles/simulink.map'], 'hmi_lamp')
      mask Display:
      | if strcmp(get_param(bdroot(gcb),'BlockDiagramType'), 'library')
      |     image([(matlabroot) '/toolbox/simulink/hmi/icons/Lamp.png']);
      | end
  Lamp51 : Subsystem  DialogController=hmiCreateDDGDialog  mask(MWDashboardBlock){webBlockId=7d3ec8dc-6aba-4c81-ba33-ed038051774f, webBlockType=lamp, ShowInLibBrowser=on, ShowInitialText=on, HMISrcModelName=[]}
      mask prompts: webBlockType "WebBlock Type"; HMISrcModelName "Source Model"
      mask Help: helpview([docroot '/mapfiles/simulink.map'], 'hmi_lamp')
      mask Display:
      | if strcmp(get_param(bdroot(gcb),'BlockDiagramType'), 'library')
      |     image([(matlabroot) '/toolbox/simulink/hmi/icons/Lamp.png']);
      | end
  Lamp52 : Subsystem  DialogController=hmiCreateDDGDialog  mask(MWDashboardBlock){webBlockId=efa0ac8c-8a00-496e-ae4c-16ef0f6defee, webBlockType=lamp, ShowInLibBrowser=on, ShowInitialText=on, HMISrcModelName=[]}
      mask prompts: webBlockType "WebBlock Type"; HMISrcModelName "Source Model"
      mask Help: helpview([docroot '/mapfiles/simulink.map'], 'hmi_lamp')
      mask Display:
      | if strcmp(get_param(bdroot(gcb),'BlockDiagramType'), 'library')
      |     image([(matlabroot) '/toolbox/simulink/hmi/icons/Lamp.png']);
      | end
  Lamp53 : Subsystem  DialogController=hmiCreateDDGDialog  mask(MWDashboardBlock){webBlockId=f352c6ba-e333-47da-9699-7540cbd117fe, webBlockType=lamp, ShowInLibBrowser=on, ShowInitialText=on, HMISrcModelName=[]}
      mask prompts: webBlockType "WebBlock Type"; HMISrcModelName "Source Model"
      mask Help: helpview([docroot '/mapfiles/simulink.map'], 'hmi_lamp')
      mask Display:
      | if strcmp(get_param(bdroot(gcb),'BlockDiagramType'), 'library')
      |     image([(matlabroot) '/toolbox/simulink/hmi/icons/Lamp.png']);
      | end
  Lamp54 : Subsystem  DialogController=hmiCreateDDGDialog  mask(MWDashboardBlock){webBlockId=460e91c6-b5a3-4ecd-968d-28757cd88c72, webBlockType=lamp, ShowInLibBrowser=on, ShowInitialText=on, HMISrcModelName=[]}
      mask prompts: webBlockType "WebBlock Type"; HMISrcModelName "Source Model"
      mask Help: helpview([docroot '/mapfiles/simulink.map'], 'hmi_lamp')
      mask Display:
      | if strcmp(get_param(bdroot(gcb),'BlockDiagramType'), 'library')
      |     image([(matlabroot) '/toolbox/simulink/hmi/icons/Lamp.png']);
      | end
  Lamp55 : Subsystem  DialogController=hmiCreateDDGDialog  mask(MWDashboardBlock){webBlockId=e7ab0fb1-2fc2-45a2-9169-a64aacb3d168, webBlockType=lamp, ShowInLibBrowser=on, ShowInitialText=on, HMISrcModelName=[]}
      mask prompts: webBlockType "WebBlock Type"; HMISrcModelName "Source Model"
      mask Help: helpview([docroot '/mapfiles/simulink.map'], 'hmi_lamp')
      mask Display:
      | if strcmp(get_param(bdroot(gcb),'BlockDiagramType'), 'library')
      |     image([(matlabroot) '/toolbox/simulink/hmi/icons/Lamp.png']);
      | end
  Lamp56 : Subsystem  DialogController=hmiCreateDDGDialog  mask(MWDashboardBlock){webBlockId=a6baf857-022f-4fcd-9186-7a9c0a18c058, webBlockType=lamp, ShowInLibBrowser=on, ShowInitialText=on, HMISrcModelName=[]}
      mask prompts: webBlockType "WebBlock Type"; HMISrcModelName "Source Model"
      mask Help: helpview([docroot '/mapfiles/simulink.map'], 'hmi_lamp')
      mask Display:
      | if strcmp(get_param(bdroot(gcb),'BlockDiagramType'), 'library')
      |     image([(matlabroot) '/toolbox/simulink/hmi/icons/Lamp.png']);
      | end
  Lamp57 : Subsystem  DialogController=hmiCreateDDGDialog  mask(MWDashboardBlock){webBlockId=56db2e4d-49b7-49c1-82ec-ee18fd0cb7b3, webBlockType=lamp, ShowInLibBrowser=on, ShowInitialText=on, HMISrcModelName=[]}
      mask prompts: webBlockType "WebBlock Type"; HMISrcModelName "Source Model"
      mask Help: helpview([docroot '/mapfiles/simulink.map'], 'hmi_lamp')
      mask Display:
      | if strcmp(get_param(bdroot(gcb),'BlockDiagramType'), 'library')
      |     image([(matlabroot) '/toolbox/simulink/hmi/icons/Lamp.png']);
      | end
  Lamp58 : Subsystem  DialogController=hmiCreateDDGDialog  mask(MWDashboardBlock){webBlockId=8bf2930a-8292-4e9d-a40b-29454ab38727, webBlockType=lamp, ShowInLibBrowser=on, ShowInitialText=on, HMISrcModelName=[]}
      mask prompts: webBlockType "WebBlock Type"; HMISrcModelName "Source Model"
      mask Help: helpview([docroot '/mapfiles/simulink.map'], 'hmi_lamp')
      mask Display:
      | if strcmp(get_param(bdroot(gcb),'BlockDiagramType'), 'library')
      |     image([(matlabroot) '/toolbox/simulink/hmi/icons/Lamp.png']);
      | end
  Lamp59 : Subsystem  DialogController=hmiCreateDDGDialog  mask(MWDashboardBlock){webBlockId=df001e5c-a79d-4f98-a834-60a4016acfe9, webBlockType=lamp, ShowInLibBrowser=on, ShowInitialText=on, HMISrcModelName=[]}
      mask prompts: webBlockType "WebBlock Type"; HMISrcModelName "Source Model"
      mask Help: helpview([docroot '/mapfiles/simulink.map'], 'hmi_lamp')
      mask Display:
      | if strcmp(get_param(bdroot(gcb),'BlockDiagramType'), 'library')
      |     image([(matlabroot) '/toolbox/simulink/hmi/icons/Lamp.png']);
      | end
  Lamp6 : Subsystem  DialogController=hmiCreateDDGDialog  mask(MWDashboardBlock){webBlockId=682566aa-b4a8-441a-af91-4aa08e41663a, webBlockType=lamp, ShowInLibBrowser=on, ShowInitialText=on, HMISrcModelName=[]}
      mask prompts: webBlockType "WebBlock Type"; HMISrcModelName "Source Model"
      mask Help: helpview([docroot '/mapfiles/simulink.map'], 'hmi_lamp')
      mask Display:
      | if strcmp(get_param(bdroot(gcb),'BlockDiagramType'), 'library')
      |     image([(matlabroot) '/toolbox/simulink/hmi/icons/Lamp.png']);
      | end
  Lamp60 : Subsystem  DialogController=hmiCreateDDGDialog  mask(MWDashboardBlock){webBlockId=2aa773e3-231c-41cc-95be-a11d281e922d, webBlockType=lamp, ShowInLibBrowser=on, ShowInitialText=on, HMISrcModelName=[]}
      mask prompts: webBlockType "WebBlock Type"; HMISrcModelName "Source Model"
      mask Help: helpview([docroot '/mapfiles/simulink.map'], 'hmi_lamp')
      mask Display:
      | if strcmp(get_param(bdroot(gcb),'BlockDiagramType'), 'library')
      |     image([(matlabroot) '/toolbox/simulink/hmi/icons/Lamp.png']);
      | end
  Lamp61 : Subsystem  DialogController=hmiCreateDDGDialog  mask(MWDashboardBlock){webBlockId=da88a90e-6267-47fa-9ffa-97270b31d1de, webBlockType=lamp, ShowInLibBrowser=on, ShowInitialText=on, HMISrcModelName=[]}
      mask prompts: webBlockType "WebBlock Type"; HMISrcModelName "Source Model"
      mask Help: helpview([docroot '/mapfiles/simulink.map'], 'hmi_lamp')
      mask Display:
      | if strcmp(get_param(bdroot(gcb),'BlockDiagramType'), 'library')
      |     image([(matlabroot) '/toolbox/simulink/hmi/icons/Lamp.png']);
      | end
  Lamp62 : Subsystem  DialogController=hmiCreateDDGDialog  mask(MWDashboardBlock){webBlockId=eee3b265-f2bc-4bdc-b529-0f4e47ee7281, webBlockType=lamp, ShowInLibBrowser=on, ShowInitialText=on, HMISrcModelName=[]}
      mask prompts: webBlockType "WebBlock Type"; HMISrcModelName "Source Model"
      mask Help: helpview([docroot '/mapfiles/simulink.map'], 'hmi_lamp')
      mask Display:
      | if strcmp(get_param(bdroot(gcb),'BlockDiagramType'), 'library')
      |     image([(matlabroot) '/toolbox/simulink/hmi/icons/Lamp.png']);
      | end
  Lamp63 : Subsystem  DialogController=hmiCreateDDGDialog  mask(MWDashboardBlock){webBlockId=a817f7d3-d3ab-4988-99d3-fbfa5d58e70c, webBlockType=lamp, ShowInLibBrowser=on, ShowInitialText=on, HMISrcModelName=[]}
      mask prompts: webBlockType "WebBlock Type"; HMISrcModelName "Source Model"
      mask Help: helpview([docroot '/mapfiles/simulink.map'], 'hmi_lamp')
      mask Display:
      | if strcmp(get_param(bdroot(gcb),'BlockDiagramType'), 'library')
      |     image([(matlabroot) '/toolbox/simulink/hmi/icons/Lamp.png']);
      | end
  Lamp64 : Subsystem  DialogController=hmiCreateDDGDialog  mask(MWDashboardBlock){webBlockId=2e55f362-185a-4bd3-b1b2-8c02f085591c, webBlockType=lamp, ShowInLibBrowser=on, ShowInitialText=on, HMISrcModelName=[]}
      mask prompts: webBlockType "WebBlock Type"; HMISrcModelName "Source Model"
      mask Help: helpview([docroot '/mapfiles/simulink.map'], 'hmi_lamp')
      mask Display:
      | if strcmp(get_param(bdroot(gcb),'BlockDiagramType'), 'library')
      |     image([(matlabroot) '/toolbox/simulink/hmi/icons/Lamp.png']);
      | end
  Lamp65 : Subsystem  DialogController=hmiCreateDDGDialog  mask(MWDashboardBlock){webBlockId=7795f2c4-47dc-446f-9f26-a50466036b34, webBlockType=lamp, ShowInLibBrowser=on, ShowInitialText=on, HMISrcModelName=[]}
      mask prompts: webBlockType "WebBlock Type"; HMISrcModelName "Source Model"
      mask Help: helpview([docroot '/mapfiles/simulink.map'], 'hmi_lamp')
      mask Display:
      | if strcmp(get_param(bdroot(gcb),'BlockDiagramType'), 'library')
      |     image([(matlabroot) '/toolbox/simulink/hmi/icons/Lamp.png']);
      | end
  Lamp66 : Subsystem  DialogController=hmiCreateDDGDialog  mask(MWDashboardBlock){webBlockId=cec75bdd-5a5f-48a6-973a-ff7b4344491d, webBlockType=lamp, ShowInLibBrowser=on, ShowInitialText=on, HMISrcModelName=[]}
      mask prompts: webBlockType "WebBlock Type"; HMISrcModelName "Source Model"
      mask Help: helpview([docroot '/mapfiles/simulink.map'], 'hmi_lamp')
      mask Display:
      | if strcmp(get_param(bdroot(gcb),'BlockDiagramType'), 'library')
      |     image([(matlabroot) '/toolbox/simulink/hmi/icons/Lamp.png']);
      | end
  Lamp67 : Subsystem  DialogController=hmiCreateDDGDialog  mask(MWDashboardBlock){webBlockId=00eb1a3f-42e1-4022-8637-a36589bd741d, webBlockType=lamp, ShowInLibBrowser=on, ShowInitialText=on, HMISrcModelName=[]}
      mask prompts: webBlockType "WebBlock Type"; HMISrcModelName "Source Model"
      mask Help: helpview([docroot '/mapfiles/simulink.map'], 'hmi_lamp')
      mask Display:
      | if strcmp(get_param(bdroot(gcb),'BlockDiagramType'), 'library')
      |     image([(matlabroot) '/toolbox/simulink/hmi/icons/Lamp.png']);
      | end
  Lamp68 : Subsystem  DialogController=hmiCreateDDGDialog  mask(MWDashboardBlock){webBlockId=705ee3cc-1626-4674-ba0a-bbd8725ba356, webBlockType=lamp, ShowInLibBrowser=on, ShowInitialText=on, HMISrcModelName=[]}
      mask prompts: webBlockType "WebBlock Type"; HMISrcModelName "Source Model"
      mask Help: helpview([docroot '/mapfiles/simulink.map'], 'hmi_lamp')
      mask Display:
      | if strcmp(get_param(bdroot(gcb),'BlockDiagramType'), 'library')
      |     image([(matlabroot) '/toolbox/simulink/hmi/icons/Lamp.png']);
      | end
  Lamp69 : Subsystem  DialogController=hmiCreateDDGDialog  mask(MWDashboardBlock){webBlockId=d10bb480-2a5f-4b5e-8e68-f02b6ba0af8d, webBlockType=lamp, ShowInLibBrowser=on, ShowInitialText=on, HMISrcModelName=[]}
      mask prompts: webBlockType "WebBlock Type"; HMISrcModelName "Source Model"
      mask Help: helpview([docroot '/mapfiles/simulink.map'], 'hmi_lamp')
      mask Display:
      | if strcmp(get_param(bdroot(gcb),'BlockDiagramType'), 'library')
      |     image([(matlabroot) '/toolbox/simulink/hmi/icons/Lamp.png']);
      | end
  Lamp7 : Subsystem  DialogController=hmiCreateDDGDialog  mask(MWDashboardBlock){webBlockId=ed87f122-f12f-4cd0-bed9-474ddf2ab17c, webBlockType=lamp, ShowInLibBrowser=on, ShowInitialText=on, HMISrcModelName=[]}
      mask prompts: webBlockType "WebBlock Type"; HMISrcModelName "Source Model"
      mask Help: helpview([docroot '/mapfiles/simulink.map'], 'hmi_lamp')
      mask Display:
      | if strcmp(get_param(bdroot(gcb),'BlockDiagramType'), 'library')
      |     image([(matlabroot) '/toolbox/simulink/hmi/icons/Lamp.png']);
      | end
  Lamp70 : Subsystem  DialogController=hmiCreateDDGDialog  mask(MWDashboardBlock){webBlockId=cdf0cc83-b1e8-4123-bb89-bbb953da003e, webBlockType=lamp, ShowInLibBrowser=on, ShowInitialText=on, HMISrcModelName=[]}
      mask prompts: webBlockType "WebBlock Type"; HMISrcModelName "Source Model"
      mask Help: helpview([docroot '/mapfiles/simulink.map'], 'hmi_lamp')
      mask Display:
      | if strcmp(get_param(bdroot(gcb),'BlockDiagramType'), 'library')
      |     image([(matlabroot) '/toolbox/simulink/hmi/icons/Lamp.png']);
      | end
  Lamp71 : Subsystem  DialogController=hmiCreateDDGDialog  mask(MWDashboardBlock){webBlockId=9f523300-f981-4e65-b343-9d2444d155c4, webBlockType=lamp, ShowInLibBrowser=on, ShowInitialText=on, HMISrcModelName=[]}
      mask prompts: webBlockType "WebBlock Type"; HMISrcModelName "Source Model"
      mask Help: helpview([docroot '/mapfiles/simulink.map'], 'hmi_lamp')
      mask Display:
      | if strcmp(get_param(bdroot(gcb),'BlockDiagramType'), 'library')
      |     image([(matlabroot) '/toolbox/simulink/hmi/icons/Lamp.png']);
      | end
  Lamp72 : Subsystem  DialogController=hmiCreateDDGDialog  mask(MWDashboardBlock){webBlockId=e8f54bdd-2a2f-4bfa-9db4-490aa2daccd4, webBlockType=lamp, ShowInLibBrowser=on, ShowInitialText=on, HMISrcModelName=[]}
      mask prompts: webBlockType "WebBlock Type"; HMISrcModelName "Source Model"
      mask Help: helpview([docroot '/mapfiles/simulink.map'], 'hmi_lamp')
      mask Display:
      | if strcmp(get_param(bdroot(gcb),'BlockDiagramType'), 'library')
      |     image([(matlabroot) '/toolbox/simulink/hmi/icons/Lamp.png']);
      | end
  Lamp73 : Subsystem  DialogController=hmiCreateDDGDialog  mask(MWDashboardBlock){webBlockId=de50a062-abaf-454b-9abb-d181155ba1cf, webBlockType=lamp, ShowInLibBrowser=on, ShowInitialText=on, HMISrcModelName=[]}
      mask prompts: webBlockType "WebBlock Type"; HMISrcModelName "Source Model"
      mask Help: helpview([docroot '/mapfiles/simulink.map'], 'hmi_lamp')
      mask Display:
      | if strcmp(get_param(bdroot(gcb),'BlockDiagramType'), 'library')
      |     image([(matlabroot) '/toolbox/simulink/hmi/icons/Lamp.png']);
      | end
  Lamp74 : Subsystem  DialogController=hmiCreateDDGDialog  mask(MWDashboardBlock){webBlockId=ce613a5b-28ea-4b44-8a0b-aa347f2b34a3, webBlockType=lamp, ShowInLibBrowser=on, ShowInitialText=on, HMISrcModelName=[]}
      mask prompts: webBlockType "WebBlock Type"; HMISrcModelName "Source Model"
      mask Help: helpview([docroot '/mapfiles/simulink.map'], 'hmi_lamp')
      mask Display:
      | if strcmp(get_param(bdroot(gcb),'BlockDiagramType'), 'library')
      |     image([(matlabroot) '/toolbox/simulink/hmi/icons/Lamp.png']);
      | end
  Lamp75 : Subsystem  DialogController=hmiCreateDDGDialog  mask(MWDashboardBlock){webBlockId=21a953f6-0877-4073-a73e-587d95f416cc, webBlockType=lamp, ShowInLibBrowser=on, ShowInitialText=on, HMISrcModelName=[]}
      mask prompts: webBlockType "WebBlock Type"; HMISrcModelName "Source Model"
      mask Help: helpview([docroot '/mapfiles/simulink.map'], 'hmi_lamp')
      mask Display:
      | if strcmp(get_param(bdroot(gcb),'BlockDiagramType'), 'library')
      |     image([(matlabroot) '/toolbox/simulink/hmi/icons/Lamp.png']);
      | end
  Lamp76 : Subsystem  DialogController=hmiCreateDDGDialog  mask(MWDashboardBlock){webBlockId=a33e02a8-e7b1-4c82-808c-cf06fae1dbc5, webBlockType=lamp, ShowInLibBrowser=on, ShowInitialText=on, HMISrcModelName=[]}
      mask prompts: webBlockType "WebBlock Type"; HMISrcModelName "Source Model"
      mask Help: helpview([docroot '/mapfiles/simulink.map'], 'hmi_lamp')
      mask Display:
      | if strcmp(get_param(bdroot(gcb),'BlockDiagramType'), 'library')
      |     image([(matlabroot) '/toolbox/simulink/hmi/icons/Lamp.png']);
      | end
  Lamp77 : Subsystem  DialogController=hmiCreateDDGDialog  mask(MWDashboardBlock){webBlockId=002bc4fa-eb90-43b8-8ae2-3456e156c15c, webBlockType=lamp, ShowInLibBrowser=on, ShowInitialText=on, HMISrcModelName=[]}
      mask prompts: webBlockType "WebBlock Type"; HMISrcModelName "Source Model"
      mask Help: helpview([docroot '/mapfiles/simulink.map'], 'hmi_lamp')
      mask Display:
      | if strcmp(get_param(bdroot(gcb),'BlockDiagramType'), 'library')
      |     image([(matlabroot) '/toolbox/simulink/hmi/icons/Lamp.png']);
      | end
  Lamp78 : Subsystem  DialogController=hmiCreateDDGDialog  mask(MWDashboardBlock){webBlockId=051994d5-643a-49e8-83a1-b7092d41aa99, webBlockType=lamp, ShowInLibBrowser=on, ShowInitialText=on, HMISrcModelName=[]}
      mask prompts: webBlockType "WebBlock Type"; HMISrcModelName "Source Model"
      mask Help: helpview([docroot '/mapfiles/simulink.map'], 'hmi_lamp')
      mask Display:
      | if strcmp(get_param(bdroot(gcb),'BlockDiagramType'), 'library')
      |     image([(matlabroot) '/toolbox/simulink/hmi/icons/Lamp.png']);
      | end
  Lamp79 : Subsystem  DialogController=hmiCreateDDGDialog  mask(MWDashboardBlock){webBlockId=616af54a-244a-4692-9d19-f50b957939d9, webBlockType=lamp, ShowInLibBrowser=on, ShowInitialText=on, HMISrcModelName=[]}
      mask prompts: webBlockType "WebBlock Type"; HMISrcModelName "Source Model"
      mask Help: helpview([docroot '/mapfiles/simulink.map'], 'hmi_lamp')
      mask Display:
      | if strcmp(get_param(bdroot(gcb),'BlockDiagramType'), 'library')
      |     image([(matlabroot) '/toolbox/simulink/hmi/icons/Lamp.png']);
      | end
  Lamp8 : Subsystem  DialogController=hmiCreateDDGDialog  mask(MWDashboardBlock){webBlockId=2cb2e590-689f-4ecb-bb1b-7cdfa7df553e, webBlockType=lamp, ShowInLibBrowser=on, ShowInitialText=on, HMISrcModelName=[]}
      mask prompts: webBlockType "WebBlock Type"; HMISrcModelName "Source Model"
      mask Help: helpview([docroot '/mapfiles/simulink.map'], 'hmi_lamp')
      mask Display:
      | if strcmp(get_param(bdroot(gcb),'BlockDiagramType'), 'library')
      |     image([(matlabroot) '/toolbox/simulink/hmi/icons/Lamp.png']);
      | end
  Lamp80 : Subsystem  DialogController=hmiCreateDDGDialog  mask(MWDashboardBlock){webBlockId=eb3997a0-55cb-48a1-93da-2023c8b36e75, webBlockType=lamp, ShowInLibBrowser=on, ShowInitialText=on, HMISrcModelName=[]}
      mask prompts: webBlockType "WebBlock Type"; HMISrcModelName "Source Model"
      mask Help: helpview([docroot '/mapfiles/simulink.map'], 'hmi_lamp')
      mask Display:
      | if strcmp(get_param(bdroot(gcb),'BlockDiagramType'), 'library')
      |     image([(matlabroot) '/toolbox/simulink/hmi/icons/Lamp.png']);
      | end
  Lamp81 : Subsystem  DialogController=hmiCreateDDGDialog  mask(MWDashboardBlock){webBlockId=aef906c7-3164-4879-93e5-072bfbe86e81, webBlockType=lamp, ShowInLibBrowser=on, ShowInitialText=on, HMISrcModelName=[]}
      mask prompts: webBlockType "WebBlock Type"; HMISrcModelName "Source Model"
      mask Help: helpview([docroot '/mapfiles/simulink.map'], 'hmi_lamp')
      mask Display:
      | if strcmp(get_param(bdroot(gcb),'BlockDiagramType'), 'library')
      |     image([(matlabroot) '/toolbox/simulink/hmi/icons/Lamp.png']);
      | end
  Lamp82 : Subsystem  DialogController=hmiCreateDDGDialog  mask(MWDashboardBlock){webBlockId=ccf6b8d2-4d9c-4614-a80c-43cf191298fe, webBlockType=lamp, ShowInLibBrowser=on, ShowInitialText=on, HMISrcModelName=[]}
      mask prompts: webBlockType "WebBlock Type"; HMISrcModelName "Source Model"
      mask Help: helpview([docroot '/mapfiles/simulink.map'], 'hmi_lamp')
      mask Display:
      | if strcmp(get_param(bdroot(gcb),'BlockDiagramType'), 'library')
      |     image([(matlabroot) '/toolbox/simulink/hmi/icons/Lamp.png']);
      | end
  Lamp83 : Subsystem  DialogController=hmiCreateDDGDialog  mask(MWDashboardBlock){webBlockId=1ee6e9ed-92ba-49b3-ad8e-271f0e0c0e55, webBlockType=lamp, ShowInLibBrowser=on, ShowInitialText=on, HMISrcModelName=[]}
      mask prompts: webBlockType "WebBlock Type"; HMISrcModelName "Source Model"
      mask Help: helpview([docroot '/mapfiles/simulink.map'], 'hmi_lamp')
      mask Display:
      | if strcmp(get_param(bdroot(gcb),'BlockDiagramType'), 'library')
      |     image([(matlabroot) '/toolbox/simulink/hmi/icons/Lamp.png']);
      | end
  Lamp84 : Subsystem  DialogController=hmiCreateDDGDialog  mask(MWDashboardBlock){webBlockId=5028fd7b-e0ec-4255-9bae-c79a4cf13ff5, webBlockType=lamp, ShowInLibBrowser=on, ShowInitialText=on, HMISrcModelName=[]}
      mask prompts: webBlockType "WebBlock Type"; HMISrcModelName "Source Model"
      mask Help: helpview([docroot '/mapfiles/simulink.map'], 'hmi_lamp')
      mask Display:
      | if strcmp(get_param(bdroot(gcb),'BlockDiagramType'), 'library')
      |     image([(matlabroot) '/toolbox/simulink/hmi/icons/Lamp.png']);
      | end
  Lamp85 : Subsystem  DialogController=hmiCreateDDGDialog  mask(MWDashboardBlock){webBlockId=013ee31d-50b7-416f-b8bc-b9d30c79ff2e, webBlockType=lamp, ShowInLibBrowser=on, ShowInitialText=on, HMISrcModelName=[]}
      mask prompts: webBlockType "WebBlock Type"; HMISrcModelName "Source Model"
      mask Help: helpview([docroot '/mapfiles/simulink.map'], 'hmi_lamp')
      mask Display:
      | if strcmp(get_param(bdroot(gcb),'BlockDiagramType'), 'library')
      |     image([(matlabroot) '/toolbox/simulink/hmi/icons/Lamp.png']);
      | end
  Lamp86 : Subsystem  DialogController=hmiCreateDDGDialog  mask(MWDashboardBlock){webBlockId=cd11274f-c078-4d73-b977-a8d93a4b28bc, webBlockType=lamp, ShowInLibBrowser=on, ShowInitialText=on, HMISrcModelName=[]}
      mask prompts: webBlockType "WebBlock Type"; HMISrcModelName "Source Model"
      mask Help: helpview([docroot '/mapfiles/simulink.map'], 'hmi_lamp')
      mask Display:
      | if strcmp(get_param(bdroot(gcb),'BlockDiagramType'), 'library')
      |     image([(matlabroot) '/toolbox/simulink/hmi/icons/Lamp.png']);
      | end
  Lamp87 : Subsystem  DialogController=hmiCreateDDGDialog  mask(MWDashboardBlock){webBlockId=4388bc0a-9699-4673-810d-2854011de202, webBlockType=lamp, ShowInLibBrowser=on, ShowInitialText=on, HMISrcModelName=[]}
      mask prompts: webBlockType "WebBlock Type"; HMISrcModelName "Source Model"
      mask Help: helpview([docroot '/mapfiles/simulink.map'], 'hmi_lamp')
      mask Display:
      | if strcmp(get_param(bdroot(gcb),'BlockDiagramType'), 'library')
      |     image([(matlabroot) '/toolbox/simulink/hmi/icons/Lamp.png']);
      | end
  Lamp88 : Subsystem  DialogController=hmiCreateDDGDialog  mask(MWDashboardBlock){webBlockId=906738bd-4550-4c6f-9401-34960625993c, webBlockType=lamp, ShowInLibBrowser=on, ShowInitialText=on, HMISrcModelName=[]}
      mask prompts: webBlockType "WebBlock Type"; HMISrcModelName "Source Model"
      mask Help: helpview([docroot '/mapfiles/simulink.map'], 'hmi_lamp')
      mask Display:
      | if strcmp(get_param(bdroot(gcb),'BlockDiagramType'), 'library')
      |     image([(matlabroot) '/toolbox/simulink/hmi/icons/Lamp.png']);
      | end
  Lamp89 : Subsystem  DialogController=hmiCreateDDGDialog  mask(MWDashboardBlock){webBlockId=0292be83-4691-4795-a960-750861d8599d, webBlockType=lamp, ShowInLibBrowser=on, ShowInitialText=on, HMISrcModelName=[]}
      mask prompts: webBlockType "WebBlock Type"; HMISrcModelName "Source Model"
      mask Help: helpview([docroot '/mapfiles/simulink.map'], 'hmi_lamp')
      mask Display:
      | if strcmp(get_param(bdroot(gcb),'BlockDiagramType'), 'library')
      |     image([(matlabroot) '/toolbox/simulink/hmi/icons/Lamp.png']);
      | end
  Lamp9 : Subsystem  DialogController=hmiCreateDDGDialog  mask(MWDashboardBlock){webBlockId=e8e3b70e-c292-4ef4-ba6e-5f59b516d004, webBlockType=lamp, ShowInLibBrowser=on, ShowInitialText=on, HMISrcModelName=[]}
      mask prompts: webBlockType "WebBlock Type"; HMISrcModelName "Source Model"
      mask Help: helpview([docroot '/mapfiles/simulink.map'], 'hmi_lamp')
      mask Display:
      | if strcmp(get_param(bdroot(gcb),'BlockDiagramType'), 'library')
      |     image([(matlabroot) '/toolbox/simulink/hmi/icons/Lamp.png']);
      | end
  Lamp90 : Subsystem  DialogController=hmiCreateDDGDialog  mask(MWDashboardBlock){webBlockId=547167c0-e93a-4166-88c4-641b49ce1af4, webBlockType=lamp, ShowInLibBrowser=on, ShowInitialText=on, HMISrcModelName=[]}
      mask prompts: webBlockType "WebBlock Type"; HMISrcModelName "Source Model"
      mask Help: helpview([docroot '/mapfiles/simulink.map'], 'hmi_lamp')
      mask Display:
      | if strcmp(get_param(bdroot(gcb),'BlockDiagramType'), 'library')
      |     image([(matlabroot) '/toolbox/simulink/hmi/icons/Lamp.png']);
      | end
  Lamp91 : Subsystem  DialogController=hmiCreateDDGDialog  mask(MWDashboardBlock){webBlockId=5c83f076-9d52-4313-bf2d-709168ba3326, webBlockType=lamp, ShowInLibBrowser=on, ShowInitialText=on, HMISrcModelName=[]}
      mask prompts: webBlockType "WebBlock Type"; HMISrcModelName "Source Model"
      mask Help: helpview([docroot '/mapfiles/simulink.map'], 'hmi_lamp')
      mask Display:
      | if strcmp(get_param(bdroot(gcb),'BlockDiagramType'), 'library')
      |     image([(matlabroot) '/toolbox/simulink/hmi/icons/Lamp.png']);
      | end
  Lamp92 : Subsystem  DialogController=hmiCreateDDGDialog  mask(MWDashboardBlock){webBlockId=da80d835-309a-4336-874c-f373f01b9747, webBlockType=lamp, ShowInLibBrowser=on, ShowInitialText=on, HMISrcModelName=[]}
      mask prompts: webBlockType "WebBlock Type"; HMISrcModelName "Source Model"
      mask Help: helpview([docroot '/mapfiles/simulink.map'], 'hmi_lamp')
      mask Display:
      | if strcmp(get_param(bdroot(gcb),'BlockDiagramType'), 'library')
      |     image([(matlabroot) '/toolbox/simulink/hmi/icons/Lamp.png']);
      | end
  Lamp93 : Subsystem  DialogController=hmiCreateDDGDialog  mask(MWDashboardBlock){webBlockId=a42d60d2-d5cb-4518-9a50-7d0f8631bd57, webBlockType=lamp, ShowInLibBrowser=on, ShowInitialText=on, HMISrcModelName=[]}
      mask prompts: webBlockType "WebBlock Type"; HMISrcModelName "Source Model"
      mask Help: helpview([docroot '/mapfiles/simulink.map'], 'hmi_lamp')
      mask Display:
      | if strcmp(get_param(bdroot(gcb),'BlockDiagramType'), 'library')
      |     image([(matlabroot) '/toolbox/simulink/hmi/icons/Lamp.png']);
      | end
  Lamp94 : Subsystem  DialogController=hmiCreateDDGDialog  mask(MWDashboardBlock){webBlockId=53c7b5ab-7957-4f99-a933-defe13551182, webBlockType=lamp, ShowInLibBrowser=on, ShowInitialText=on, HMISrcModelName=[]}
      mask prompts: webBlockType "WebBlock Type"; HMISrcModelName "Source Model"
      mask Help: helpview([docroot '/mapfiles/simulink.map'], 'hmi_lamp')
      mask Display:
      | if strcmp(get_param(bdroot(gcb),'BlockDiagramType'), 'library')
      |     image([(matlabroot) '/toolbox/simulink/hmi/icons/Lamp.png']);
      | end
  Lamp95 : Subsystem  DialogController=hmiCreateDDGDialog  mask(MWDashboardBlock){webBlockId=b8d9fd2f-bf3c-48f1-bb4b-1f66f1c14b80, webBlockType=lamp, ShowInLibBrowser=on, ShowInitialText=on, HMISrcModelName=[]}
      mask prompts: webBlockType "WebBlock Type"; HMISrcModelName "Source Model"
      mask Help: helpview([docroot '/mapfiles/simulink.map'], 'hmi_lamp')
      mask Display:
      | if strcmp(get_param(bdroot(gcb),'BlockDiagramType'), 'library')
      |     image([(matlabroot) '/toolbox/simulink/hmi/icons/Lamp.png']);
      | end
  Lamp96 : Subsystem  DialogController=hmiCreateDDGDialog  mask(MWDashboardBlock){webBlockId=ad1324e1-9945-4136-9dbb-85947771c1c8, webBlockType=lamp, ShowInLibBrowser=on, ShowInitialText=on, HMISrcModelName=[]}
      mask prompts: webBlockType "WebBlock Type"; HMISrcModelName "Source Model"
      mask Help: helpview([docroot '/mapfiles/simulink.map'], 'hmi_lamp')
      mask Display:
      | if strcmp(get_param(bdroot(gcb),'BlockDiagramType'), 'library')
      |     image([(matlabroot) '/toolbox/simulink/hmi/icons/Lamp.png']);
      | end
  Lamp97 : Subsystem  DialogController=hmiCreateDDGDialog  mask(MWDashboardBlock){webBlockId=db8ebaf0-d883-494e-942d-761864daad52, webBlockType=lamp, ShowInLibBrowser=on, ShowInitialText=on, HMISrcModelName=[]}
      mask prompts: webBlockType "WebBlock Type"; HMISrcModelName "Source Model"
      mask Help: helpview([docroot '/mapfiles/simulink.map'], 'hmi_lamp')
      mask Display:
      | if strcmp(get_param(bdroot(gcb),'BlockDiagramType'), 'library')
      |     image([(matlabroot) '/toolbox/simulink/hmi/icons/Lamp.png']);
      | end
  Lamp98 : Subsystem  DialogController=hmiCreateDDGDialog  mask(MWDashboardBlock){webBlockId=83e71879-5469-4a6b-8a6c-38211729bc6f, webBlockType=lamp, ShowInLibBrowser=on, ShowInitialText=on, HMISrcModelName=[]}
      mask prompts: webBlockType "WebBlock Type"; HMISrcModelName "Source Model"
      mask Help: helpview([docroot '/mapfiles/simulink.map'], 'hmi_lamp')
      mask Display:
      | if strcmp(get_param(bdroot(gcb),'BlockDiagramType'), 'library')
      |     image([(matlabroot) '/toolbox/simulink/hmi/icons/Lamp.png']);
      | end
  Lamp99 : Subsystem  DialogController=hmiCreateDDGDialog  mask(MWDashboardBlock){}
      mask Help: helpview([docroot '/mapfiles/simulink.map'], 'hmi_lamp')
      mask Display:
      | if strcmp(get_param(bdroot(gcb),'BlockDiagramType'), 'library')
      |     image([(matlabroot) '/toolbox/simulink/hmi/icons/Lamp.png']);
      | end
